simulink model "FreeFloatingNull"  (R2019a)
settings: Solver=VariableStepAuto  StartTime=0.0  StopTime=30  RelTol=1e-3
values from neighbouring files (symbols this model uses):
  deltaQdotGainArm = 1    [main.m]
  eePositionGain = 3    [main.m]
  eeVelocityGain = 1    [main.m]
  qJoints_init = [0; -0.5236; 0; -1.0472; 0; -1.0472; 0]    [main.m]
undefined symbols (not defined in the file or in its folder): sigbuilder_block, X, Y, Z
libraries: sm_lib x99, nesl_utility x51, robotcorelib x4, simulink_extras x1
(part 1 of 3)
settings Model: Creator=tori  LastModifiedBy=tori

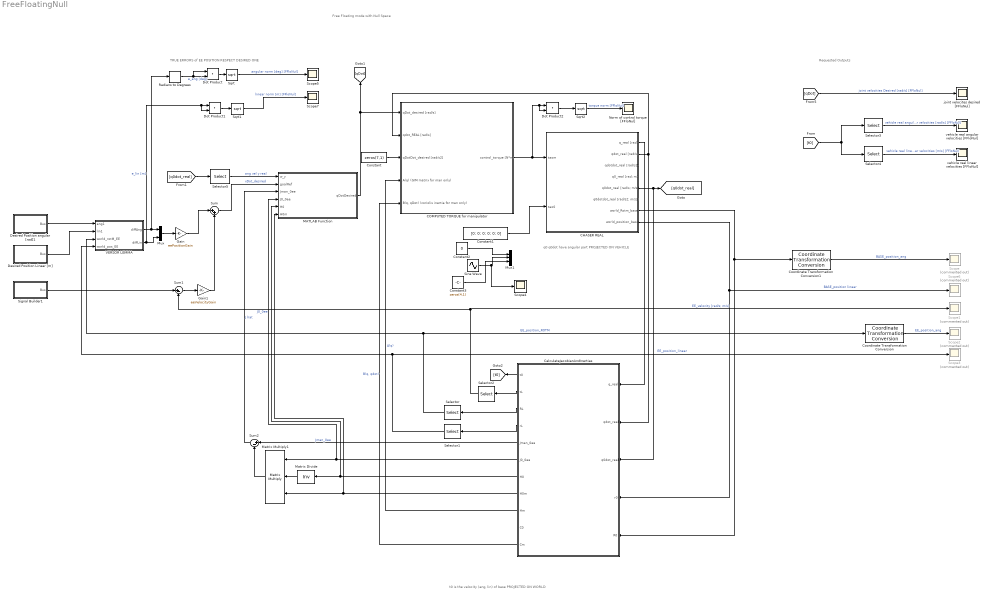
== system FreeFloatingNull ==
  note: q0 q0dot have angular part PROJECTED ON VEHICLE
  note: t0 is the velocity (ang, lin) of base PROJECTED ON WORLD
  note: TRUE ERRORS of EE POSITION RESPECT DESIRED ONE
  note: Free Floating mode with Null Space
  note: Requested Outputs
  "CHASER REAL " : Subsystem
  COMPUTED TORQUE for manipulator : Subsystem  mask{deltaQdotGainArm_int=deltaQdotGainArm}
      mask prompts: deltaQdotGainArm_int "Gain for deltaQdot"
  CalculateJacobianAndInertias : MATLAB Function  TreatAsAtomicUnit=on
  Constant : Constant  Value=zeros(7,1)
  Constant1 : Constant  Value=[0; 0; 0; 0; 0; 0]
  Constant2 : Constant  Value=0
  Constant3 : Constant  Value=zeros(4,1)
  Coordinate Transformation Conversion : robotcorelib/Coordinate Transformation Conversion  InputRepresentation=Rotation Matrix  InputEulerSequence=ZYX  ShowTrVecInputPort=on  OutputRepresentation=Euler Angles  OutputEulerSequence=ZYX  ShowTrVecOutputPort=on  SimulateUsing=Interpreted execution
      settings: SourceProductBaseCode=RO
  Coordinate Transformation Conversion1 : robotcorelib/Coordinate Transformation Conversion  InputRepresentation=Rotation Matrix  InputEulerSequence=ZYX  ShowTrVecInputPort=on  OutputRepresentation=Euler Angles  OutputEulerSequence=ZYX  ShowTrVecOutputPort=on  SimulateUsing=Interpreted execution
      settings: SourceProductBaseCode=RO
  "Desired Position Linear [m] " : Subsystem  Tag=STV Subsys  LoadFcn=sigbuilder_block('load');  StartFcn=sigbuilder_block('start');  StopFcn=sigbuilder_block('stop');  ClipboardFcn=sigbuilder_block('clipboard');  mask(Sigbuilder block){tuvar=[0:10]}
      mask help: Simulink:masks:SigbuilderBlock_MD
      mask init:
      | if ~strcmp(get_param(bdroot(gcbh),'SimulationStatus'),'stopped') tuvar = sigbuilder_block('maskInit'); end
      settings: CopyFcn=sigbuilder_block('copy');  DeleteFcn=sigbuilder_block('delete');  ModelCloseFcn=sigbuilder_block('modelClose');  PreSaveFcn=sigbuilder_block('preSave');  PauseFcn=sigbuilder_block('pause');  ContinueFcn=sigbuilder_block('continue');  NameChangeFcn=sigbuilder_block('namechange');  OpenFcn=sigbuilder_block('open',[4.5 0 1432.5 645.75 ]);  CloseFcn=sigbuilder_block('close');
      mask Display: plot(0, 0, 100, 100,[2, 2, 32, 32, 2], [68, 8, 8, 68, 68],[32, 2], [38, 38], [32, 19, 2],[53, 60, 44], [32, 17, 17, 2],[16, 16, 31, 31]);txt = getActiveGroup(gcbh);text(2, 100, txt,'verticalAlignment', 'top');
  Desired Position angular [rad]1 : Subsystem  Tag=STV Subsys  LoadFcn=sigbuilder_block('load');  StartFcn=sigbuilder_block('start');  StopFcn=sigbuilder_block('stop');  ClipboardFcn=sigbuilder_block('clipboard');  mask(Sigbuilder block){tuvar=[0:10]}
      mask help: Simulink:masks:SigbuilderBlock_MD
      mask init:
      | if ~strcmp(get_param(bdroot(gcbh),'SimulationStatus'),'stopped') tuvar = sigbuilder_block('maskInit'); end
      settings: CopyFcn=sigbuilder_block('copy');  DeleteFcn=sigbuilder_block('delete');  ModelCloseFcn=sigbuilder_block('modelClose');  PreSaveFcn=sigbuilder_block('preSave');  PauseFcn=sigbuilder_block('pause');  ContinueFcn=sigbuilder_block('continue');  NameChangeFcn=sigbuilder_block('namechange');  OpenFcn=sigbuilder_block('open',[0 0 1440 589.5 ]);  CloseFcn=sigbuilder_block('close');
      mask Display: plot(0, 0, 100, 100,[2, 2, 32, 32, 2], [68, 8, 8, 68, 68],[32, 2], [38, 38], [32, 19, 2],[53, 60, 44], [32, 17, 17, 2],[16, 16, 31, 31]);txt = getActiveGroup(gcbh);text(2, 100, txt,'verticalAlignment', 'top');
  Dot Product : DotProduct  InputSameDT=on  OutDataTypeStr=Inherit: Inherit via internal rule
  Dot Product1 : DotProduct  InputSameDT=on  OutDataTypeStr=Inherit: Inherit via internal rule
  Dot Product2 : DotProduct  InputSameDT=on  OutDataTypeStr=Inherit: Inherit via internal rule
  Gain : Gain  Gain=eePositionGain
  Gain1 : Gain  Gain=eeVelocityGain
  MATLAB Function : MATLAB Function  TreatAsAtomicUnit=on
  Matrix Divide : Product  Inputs=/  Multiplication=Matrix(*)
  Matrix Multiply1 : Product  Inputs=3  Multiplication=Matrix(*)
  Mux : Mux  Inputs=2
  Mux1 : Mux  Inputs=3
  Norm of control torque [FFloNul] : Scope
  Radians to Degrees : simulink_extras/Transformations/Radians to Degrees
  Scope{,1..3,6} (5 alike) : Scope  Commented=on
  Scope4 : Scope
  Scope5 : Scope
  Scope7 : Scope
  Selector : Selector  NumberOfDimensions=3  InputPortWidth=3  IndexOptions=Select all,Select all,Starting index (dialog)  Indices=[1 3],1,8  OutputSizes=1,1,1
  Selector1 : Selector  NumberOfDimensions=2  InputPortWidth=3  IndexOptions=Select all,Starting index (dialog)  Indices=[1 3],8  OutputSizes=1,1
  Selector2 : Selector  NumberOfDimensions=2  InputPortWidth=3  IndexOptions=Select all,Starting index (dialog)  Indices=[1 3],8  OutputSizes=1,1
  Selector3 : Selector  InputPortWidth=6  IndexOptions=Index vector (dialog)  Indices=[1 2 3]  OutputSizes=1
  Selector4 : Selector  InputPortWidth=6  IndexOptions=Index vector (dialog)  Indices=[4 5 6]  OutputSizes=1
  Selector5 : Selector  InputPortWidth=6  IndexOptions=Index vector (dialog)  Indices=[2]  OutputSizes=1
  Signal Builder1 : Subsystem  Tag=STV Subsys  LoadFcn=sigbuilder_block('load');  StartFcn=sigbuilder_block('start');  StopFcn=sigbuilder_block('stop');  ClipboardFcn=sigbuilder_block('clipboard');  mask(Sigbuilder block){tuvar=[0:10]}
      mask help: Simulink:masks:SigbuilderBlock_MD
      mask init:
      | if ~strcmp(get_param(bdroot(gcbh),'SimulationStatus'),'stopped') tuvar = sigbuilder_block('maskInit'); end
      settings: CopyFcn=sigbuilder_block('copy');  DeleteFcn=sigbuilder_block('delete');  ModelCloseFcn=sigbuilder_block('modelClose');  PreSaveFcn=sigbuilder_block('preSave');  PauseFcn=sigbuilder_block('pause');  ContinueFcn=sigbuilder_block('continue');  NameChangeFcn=sigbuilder_block('namechange');  OpenFcn=sigbuilder_block('open',[8.25 0 720 724.5 ]);  CloseFcn=sigbuilder_block('close');
      mask Display: plot(0, 0, 100, 100,[2, 2, 32, 32, 2], [68, 8, 8, 68, 68],[32, 2], [38, 38], [32, 19, 2],[53, 60, 44], [32, 17, 17, 2],[16, 16, 31, 31]);txt = getActiveGroup(gcbh);text(2, 100, txt,'verticalAlignment', 'top');
  Sine Wave : Sin  Amplitude=10  SampleTime=0
  Sqrt : Sqrt  SaturateOnIntegerOverflow=on
  Sqrt1 : Sqrt  SaturateOnIntegerOverflow=on
  Sqrt2 : Sqrt  SaturateOnIntegerOverflow=on
  Sum : Sum  Inputs=|++
  Sum1 : Sum  Inputs=|+-
  Sum2 : Sum  Inputs=|+-
  VERSOR LEMMA : MATLAB Function  TreatAsAtomicUnit=on
  "joint velocites desired [FFloNul] " : Scope
  vehicle real angular velocities [FFloNul] : Scope
  vehicle real linear velocities [FFloNul] : Scope
  wires:
  CalculateJacobianAndInertias/4(rL) -> Selector1/1
  Selector/1 -> Coordinate Transformation Conversion/1, VERSOR LEMMA/3(world_rotM_EE)  "EE_position_ROTM"
  CalculateJacobianAndInertias/9(Hm) -> COMPUTED TORQUE for manipulator/4(A(q) (GIM matrix for man only))  "A(q)"
  VERSOR LEMMA/2(diffLin) -> Dot Product1/2, Dot Product1/1, Mux/2  "e_lin [m]"
  CalculateJacobianAndInertias/11(Cm) -> COMPUTED TORQUE for manipulator/5("B(q, qDot) (coriolis inertia for man only)")  "B(q, qdot)"
  "Desired Position Linear [m] "/1(Bus) -> VERSOR LEMMA/2(lin1)
  Sum1/1 -> Gain1/1
  "CHASER REAL "/1(q_real [rad]) -> CalculateJacobianAndInertias/1(q_real)
  CalculateJacobianAndInertias/2(tL) -> Selector2/1
  Selector4/1 -> vehicle real linear velocities [FFloNul]/1  "vehicle real linear velocities [m/s] [FFloNul]"
  Sum/1 -> MATLAB Function/2(goalRef)  "xDot_desired"
  Selector3/1 -> vehicle real angular velocities [FFloNul]/1  "vehicle real angular velocities [rad/s] [FFloNul]"
  "CHASER REAL "/7("world_Rotm_base ") -> CalculateJacobianAndInertias/5(R0), Coordinate Transformation Conversion1/1
  VERSOR LEMMA/1(diffAng) -> Radians to Degrees/1, Mux/1
  Coordinate Transformation Conversion/1 -> Scope2/1  "EE_position_ang"
  Gain1/1 -> Sum/2
  Selector2/1 -> Sum1/2, Scope1/1  "EE_velocity [rad/s; m/s]"
  "CHASER REAL "/8(world_position_base) -> CalculateJacobianAndInertias/4(r0), Scope6/1  "BASE_position linear"
  [qDot] -> "joint velocites desired [FFloNul] "/1  "joint velocities Desired [rad/s] [FFloNul]"
  Signal Builder1/1(Bus) -> Sum1/1
  Mux/1 -> Gain/1
  Desired Position angular [rad]1/1(Bus) -> VERSOR LEMMA/1(ang1)
  Radians to Degrees/1 -> Dot Product/2, Dot Product/1  "e_ang [deg]"
  Constant/1 -> COMPUTED TORQUE for manipulator/3(qDotDot_desired [rad/s2])
  Selector1/1 -> Scope3/1, VERSOR LEMMA/4(world_pos_EE)  "EE_position_linear"
  Coordinate Transformation Conversion1/1 -> Scope/1  "BASE_position_ang"
  [t0] -> Selector4/1, Selector3/1
  Gain/1 -> Sum/1
  "CHASER REAL "/5(q0dot_real [rad/s; m/s]) -> [q0dot_real], CalculateJacobianAndInertias/3(q0dot_real)
  "CHASER REAL "/2(qdot_real [rad/s]) -> COMPUTED TORQUE for manipulator/2(qdot_REAL [rad/s]), CalculateJacobianAndInertias/2(qdot_real)
  CalculateJacobianAndInertias/3(RL) -> Selector/1
  Selector5/1 -> MATLAB Function/1(w_y)  "ang vel y real"
  Sqrt/1 -> Scope5/1  "angular norm [deg] [FFloNul]"
  Dot Product/1 -> Sqrt/1
  Dot Product1/1 -> Sqrt1/1
  Sqrt1/1 -> Scope7/1  "linear norm [m] [FFloNul]"
  Sqrt2/1 -> Norm of control torque [FFloNul]/1  "torque norm [FFloNul]"
  COMPUTED TORQUE for manipulator/1(control_torque [N*m]) -> Dot Product2/2, Dot Product2/1, "CHASER REAL "/1("taom ")
  Dot Product2/1 -> Sqrt2/1
  Sine Wave/1 -> Scope4/1, Mux1/2
  Constant2/1 -> Mux1/1
  Constant3/1 -> Mux1/3
  Sum2/1 -> MATLAB Function/3(Jman_0ee)  "J hat"
  CalculateJacobianAndInertias/5(Jman_0ee) -> Sum2/1  "Jman_0ee"
  CalculateJacobianAndInertias/7(H0) -> MATLAB Function/5(H0), Matrix Divide/1
  Matrix Divide/1 -> Matrix Multiply1/2
  CalculateJacobianAndInertias/8(H0m) -> MATLAB Function/6(H0m), Matrix Multiply1/3
  Matrix Multiply1/1 -> Sum2/2
  MATLAB Function/1(qDotDesired) -> COMPUTED TORQUE for manipulator/1(qDot_desired [rad/s]), [qDot]
  CalculateJacobianAndInertias/1(t0) -> [t0]
  CalculateJacobianAndInertias/6(J0_0ee) -> MATLAB Function/4(J0_0ee), Matrix Multiply1/1  "J0_0ee"
  [q0dot_real] -> Selector5/1
  Constant1/1 -> "CHASER REAL "/2(tao0)

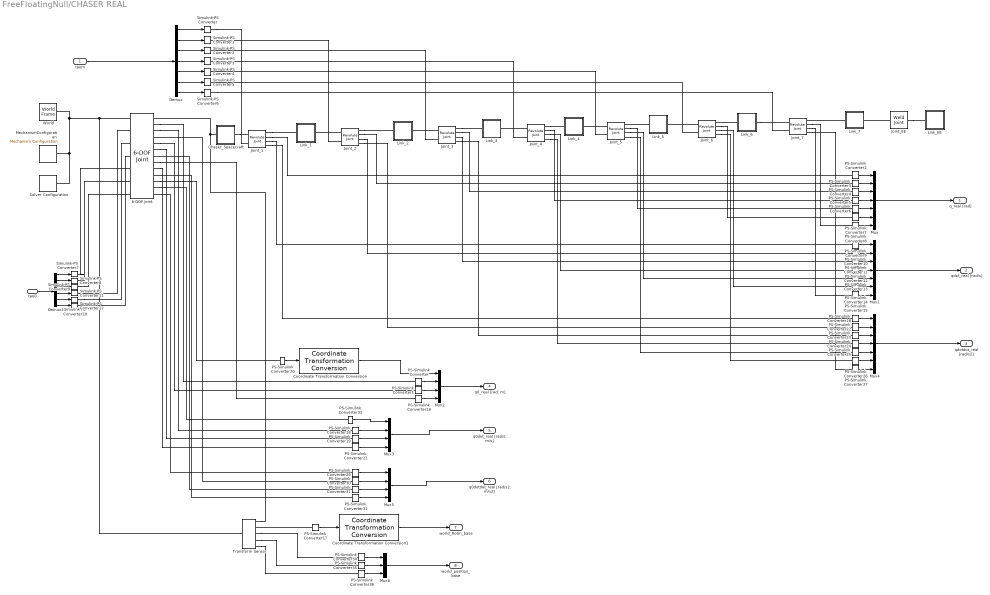
== system FreeFloatingNull/CHASER REAL  ==
  "taom " : Inport
  tao0 : Inport  Port=2
  6-DOF Joint : sm_lib/Joints/6-DOF Joint  SenseConstraintForce=off  SenseConstraintForceX=off  SenseConstraintForceY=off  SenseConstraintForceZ=off  SenseConstraintTorque=off  SenseConstraintTorqueX=off  SenseConstraintTorqueY=off  SenseConstraintTorqueZ=off  SenseTotalForce=off  SenseTotalForceX=off  SenseTotalForceY=off  SenseTotalForceZ=off  SenseTotalTorque=off  SenseTotalTorqueX=off  SenseTotalTorqueY=off  SenseTotalTorqueZ=off  CompositeWrenchDir=FollowerOnBase  CompositeWrenchFrame=BaseFrame  PxEquilibriumPosition=0  PxEquilibriumPositionUnits=m  PxSpringStiffness=0  PxSpringStiffnessUnits=N/m  PxDampingCoefficient=0  PxDampingCoefficientUnits=N/(m/s)  PxTorqueActuationMode=InputTorque  PxMotionActuationMode=ComputedMotion  PxSensePosition=on  PxSenseVelocity=on  PxSenseAcceleration=on  PxSenseTorqueForce=off  PxSenseLowerLimitTorqueForce=off  PxSenseUpperLimitTorqueForce=off  PxLowerLimitSpecify=off  PxLowerLimitBound=-1  PxLowerLimitBoundUnits=m  PxLowerLimitStiffness=1e6  PxLowerLimitStiffnessUnits=N/m  PxLowerLimitDamping=1e3  PxLowerLimitDampingUnits=N/(m/s)  PxLowerLimitTransitionRegionWidth=1e-4  PxLowerLimitTransitionRegionWidthUnits=m  PxUpperLimitSpecify=off  PxUpperLimitBound=1  PxUpperLimitBoundUnits=m  PxUpperLimitStiffness=1e6  PxUpperLimitStiffnessUnits=N/m  PxUpperLimitDamping=1e3  PxUpperLimitDampingUnits=N/(m/s)  PxUpperLimitTransitionRegionWidth=1e-4  PxUpperLimitTransitionRegionWidthUnits=m  PxPositionTargetSpecify=off  PxPositionTargetPriority=High  PxPositionTargetValue=0  PxPositionTargetValueUnits=m  PxVelocityTargetSpecify=off  PxVelocityTargetPriority=High  PxVelocityTargetValue=0  PxVelocityTargetValueUnits=m/s  PyEquilibriumPosition=0  PyEquilibriumPositionUnits=m  PySpringStiffness=0  PySpringStiffnessUnits=N/m  PyDampingCoefficient=0  PyDampingCoefficientUnits=N/(m/s)  PyTorqueActuationMode=InputTorque  PyMotionActuationMode=ComputedMotion  PySensePosition=on  PySenseVelocity=on  PySenseAcceleration=on  PySenseTorqueForce=off  PySenseLowerLimitTorqueForce=off  PySenseUpperLimitTorqueForce=off  PyLowerLimitSpecify=off  PyLowerLimitBound=-1  PyLowerLimitBoundUnits=m  PyLowerLimitStiffness=1e6  PyLowerLimitStiffnessUnits=N/m  PyLowerLimitDamping=1e3  PyLowerLimitDampingUnits=N/(m/s)  PyLowerLimitTransitionRegionWidth=1e-4  PyLowerLimitTransitionRegionWidthUnits=m  PyUpperLimitSpecify=off  PyUpperLimitBound=1  PyUpperLimitBoundUnits=m  PyUpperLimitStiffness=1e6  PyUpperLimitStiffnessUnits=N/m  PyUpperLimitDamping=1e3  PyUpperLimitDampingUnits=N/(m/s)  PyUpperLimitTransitionRegionWidth=1e-4  PyUpperLimitTransitionRegionWidthUnits=m  PyPositionTargetSpecify=off  PyPositionTargetPriority=High  PyPositionTargetValue=0  PyPositionTargetValueUnits=m  PyVelocityTargetSpecify=off  PyVelocityTargetPriority=High  PyVelocityTargetValue=0  PyVelocityTargetValueUnits=m/s  PzEquilibriumPosition=0  PzEquilibriumPositionUnits=m  PzSpringStiffness=0  PzSpringStiffnessUnits=N/m  PzDampingCoefficient=0  PzDampingCoefficientUnits=N/(m/s)  PzTorqueActuationMode=InputTorque  PzMotionActuationMode=ComputedMotion  PzSensePosition=on  PzSenseVelocity=on  PzSenseAcceleration=on  PzSenseTorqueForce=off  PzSenseLowerLimitTorqueForce=off  PzSenseUpperLimitTorqueForce=off  PzLowerLimitSpecify=off  PzLowerLimitBound=-1  PzLowerLimitBoundUnits=m  PzLowerLimitStiffness=1e6  PzLowerLimitStiffnessUnits=N/m  PzLowerLimitDamping=1e3  PzLowerLimitDampingUnits=N/(m/s)  PzLowerLimitTransitionRegionWidth=1e-4  PzLowerLimitTransitionRegionWidthUnits=m  PzUpperLimitSpecify=off  PzUpperLimitBound=1  PzUpperLimitBoundUnits=m  PzUpperLimitStiffness=1e6  PzUpperLimitStiffnessUnits=N/m  PzUpperLimitDamping=1e3  PzUpperLimitDampingUnits=N/(m/s)  PzUpperLimitTransitionRegionWidth=1e-4  PzUpperLimitTransitionRegionWidthUnits=m  PzPositionTargetSpecify=off  PzPositionTargetPriority=High  PzPositionTargetValue=0  PzPositionTargetValueUnits=m  PzVelocityTargetSpecify=off  PzVelocityTargetPriority=High  PzVelocityTargetValue=0  PzVelocityTargetValueUnits=m/s  SphDefPosRotationMethod=None  SphDefPosRotationAngleUnits=deg  SphDefPosRotationStandardAxis=+Z  SphDefPosRotationAngle=0.0  SphDefPosRotationArbitraryAxis=[0 0 1]  SphDefPosFollAlignAxisA=+X  SphDefPosBaseAlignAxisA=+Y  SphDefPosFollAlignAxisB=+Y  SphDefPosBaseAlignAxisB=+Z  SphDefPosRotationSequenceAxes=FollowerAxes  SphDefPosRotationSequence=XYX  SphDefPosRotationSequenceAngles=[0 0 0]  SphDefPosRotationSequenceAnglesUnits=deg  SphDefPosRotationMatrix=[1 0 0; 0 1 0; 0 0 1]  SphEqPosRotationMethod=None  SphEqPosRotationAngleUnits=deg  SphEqPosRotationStandardAxis=+Z  SphEqPosRotationAngle=0.0  SphEqPosRotationArbitraryAxis=[0 0 1]  SphEqPosFollAlignAxisA=+X  SphEqPosBaseAlignAxisA=+Y  SphEqPosFollAlignAxisB=+Y  SphEqPosBaseAlignAxisB=+Z  SphEqPosRotationSequenceAxes=FollowerAxes  SphEqPosRotationSequence=XYX  SphEqPosRotationSequenceAngles=[0 0 0]  SphEqPosRotationSequenceAnglesUnits=deg  SphEqPosRotationMatrix=[1 0 0; 0 1 0; 0 0 1]  SphSpringStiffness=0  SphSpringStiffnessUnits=N*m/deg  SphDampingCoefficient=0  SphDampingCoefficientUnits=N*m/(deg/s)  SphActuateTorqueX=on  SphActuateTorqueY=on  SphActuateTorqueZ=on  SphActuateTorque=off  SphTorqueActuationMode=InputTorque  SphMotionActuationMode=ComputedMotion  SphActuationFrame=FollowerFrame  SphSensePosition=on  SphSenseVelocityX=off  SphSenseVelocityY=off  SphSenseVelocityZ=off  SphSenseVelocity=on  SphSenseAccelerationX=off  SphSenseAccelerationY=off  SphSenseAccelerationZ=off  SphSenseAcceleration=on  SphSenseTorqueX=off  SphSenseTorqueY=off  SphSenseTorqueZ=off  SphSenseTorqueForce=off  SphSenseLowerLimitTorqueMag=off  SphSenseUpperLimitTorqueMag=off  SphSensingFrame=FollowerFrame  SphLowerLimitSpecify=off  SphLowerLimitBound=15  SphLowerLimitBoundUnits=deg  SphLowerLimitStiffness=1e4  SphLowerLimitStiffnessUnits=N*m/deg  SphLowerLimitDamping=10  SphLowerLimitDampingUnits=N*m/(deg/s)  SphLowerLimitTransitionRegionWidth=0.1  SphLowerLimitTransitionRegionWidthUnits=deg  SphUpperLimitSpecify=off  SphUpperLimitBound=45  SphUpperLimitBoundUnits=deg  SphUpperLimitStiffness=1e4  SphUpperLimitStiffnessUnits=N*m/deg  SphUpperLimitDamping=10  SphUpperLimitDampingUnits=N*m/(deg/s)  SphUpperLimitTransitionRegionWidth=0.1  SphUpperLimitTransitionRegionWidthUnits=deg  SphPositionTargetRotationMethod=None  SphPositionTargetRotationAngleUnits=deg  SphPositionTargetRotationStandardAxis=+Z  SphPositionTargetRotationAngle=0.0  SphPositionTargetRotationArbitraryAxis=[0 0 1]  SphPositionTargetFollAlignAxisA=+X  SphPositionTargetBaseAlignAxisA=+Y  SphPositionTargetFollAlignAxisB=+Y  SphPositionTargetBaseAlignAxisB=+Z  SphPositionTargetRotationSequenceAxes=FollowerAxes  SphPositionTargetRotationSequence=XYX  SphPositionTargetRotationSequenceAngles=[0 0 0]  SphPositionTargetRotationSequenceAnglesUnits=deg  SphPositionTargetRotationMatrix=[1 0 0; 0 1 0; 0 0 1]  SphPositionTargetSpecify=off  SphPositionTargetPriority=High  SphVelocityTargetValue=[0 0 0]  SphVelocityTargetValueUnits=deg/s  SphVelocityTargetSpecify=off  SphVelocityTargetPriority=High  SphVelocityTargetInFollowerFrame=on
  Chaser_Spacecraft : Subsystem
  Coordinate Transformation Conversion : robotcorelib/Coordinate Transformation Conversion  InputRepresentation=Quaternion  InputEulerSequence=ZYX  ShowTrVecInputPort=on  OutputRepresentation=Euler Angles  OutputEulerSequence=ZYX  ShowTrVecOutputPort=on  SimulateUsing=Interpreted execution
      settings: SourceProductBaseCode=RO
  Coordinate Transformation Conversion1 : robotcorelib/Coordinate Transformation Conversion  InputRepresentation=Quaternion  InputEulerSequence=ZYX  ShowTrVecInputPort=on  OutputRepresentation=Rotation Matrix  OutputEulerSequence=ZYX  ShowTrVecOutputPort=on  SimulateUsing=Interpreted execution
      settings: SourceProductBaseCode=RO
  Demux : Demux  Outputs=7
  Demux1 : Demux  Outputs=6
  Joint_1 : sm_lib/Joints/Revolute Joint  SenseConstraintForce=off  SenseConstraintForceX=off  SenseConstraintForceY=off  SenseConstraintForceZ=off  SenseConstraintTorque=off  SenseConstraintTorqueX=off  SenseConstraintTorqueY=off  SenseConstraintTorqueZ=off  SenseTotalForce=off  SenseTotalForceX=off  SenseTotalForceY=off  SenseTotalForceZ=off  SenseTotalTorque=off  SenseTotalTorqueX=off  SenseTotalTorqueY=off  SenseTotalTorqueZ=off  CompositeWrenchDir=FollowerOnBase  CompositeWrenchFrame=BaseFrame  EquilibriumPosition=0  EquilibriumPositionUnits=deg  SpringStiffness=0  SpringStiffnessUnits=N*m/deg  DampingCoefficient=0  DampingCoefficientUnits=m^2*kg/s/rad  TorqueActuationMode=InputTorque  MotionActuationMode=ComputedMotion  SensePosition=on  SenseVelocity=on  SenseAcceleration=on  SenseTorqueForce=off  SenseLowerLimitTorqueForce=off  SenseUpperLimitTorqueForce=off  LowerLimitSpecify=off  LowerLimitBound=-90  LowerLimitBoundUnits=deg  LowerLimitStiffness=1e4  LowerLimitStiffnessUnits=N*m/deg  LowerLimitDamping=10  LowerLimitDampingUnits=N*m/(deg/s)  LowerLimitTransitionRegionWidth=0.1  LowerLimitTransitionRegionWidthUnits=deg  UpperLimitSpecify=off  UpperLimitBound=90  UpperLimitBoundUnits=deg  UpperLimitStiffness=1e4  UpperLimitStiffnessUnits=N*m/deg  UpperLimitDamping=10  UpperLimitDampingUnits=N*m/(deg/s)  UpperLimitTransitionRegionWidth=0.1  UpperLimitTransitionRegionWidthUnits=deg  PositionTargetSpecify=on  PositionTargetPriority=High  PositionTargetValue=qJoints_init(1)  PositionTargetValueUnits=rad  VelocityTargetSpecify=off  VelocityTargetPriority=High  VelocityTargetValue=0  VelocityTargetValueUnits=deg/s
  Joint_2 : sm_lib/Joints/Revolute Joint  SenseConstraintForce=off  SenseConstraintForceX=off  SenseConstraintForceY=off  SenseConstraintForceZ=off  SenseConstraintTorque=off  SenseConstraintTorqueX=off  SenseConstraintTorqueY=off  SenseConstraintTorqueZ=off  SenseTotalForce=off  SenseTotalForceX=off  SenseTotalForceY=off  SenseTotalForceZ=off  SenseTotalTorque=off  SenseTotalTorqueX=off  SenseTotalTorqueY=off  SenseTotalTorqueZ=off  CompositeWrenchDir=FollowerOnBase  CompositeWrenchFrame=BaseFrame  EquilibriumPosition=0  EquilibriumPositionUnits=deg  SpringStiffness=0  SpringStiffnessUnits=N*m/deg  DampingCoefficient=0  DampingCoefficientUnits=m^2*kg/s/rad  TorqueActuationMode=InputTorque  MotionActuationMode=ComputedMotion  SensePosition=on  SenseVelocity=on  SenseAcceleration=on  SenseTorqueForce=off  SenseLowerLimitTorqueForce=off  SenseUpperLimitTorqueForce=off  LowerLimitSpecify=off  LowerLimitBound=-90  LowerLimitBoundUnits=deg  LowerLimitStiffness=1e4  LowerLimitStiffnessUnits=N*m/deg  LowerLimitDamping=10  LowerLimitDampingUnits=N*m/(deg/s)  LowerLimitTransitionRegionWidth=0.1  LowerLimitTransitionRegionWidthUnits=deg  UpperLimitSpecify=off  UpperLimitBound=90  UpperLimitBoundUnits=deg  UpperLimitStiffness=1e4  UpperLimitStiffnessUnits=N*m/deg  UpperLimitDamping=10  UpperLimitDampingUnits=N*m/(deg/s)  UpperLimitTransitionRegionWidth=0.1  UpperLimitTransitionRegionWidthUnits=deg  PositionTargetSpecify=on  PositionTargetPriority=High  PositionTargetValue=qJoints_init(2)  PositionTargetValueUnits=rad  VelocityTargetSpecify=off  VelocityTargetPriority=High  VelocityTargetValue=0  VelocityTargetValueUnits=deg/s
  Joint_3 : sm_lib/Joints/Revolute Joint  SenseConstraintForce=off  SenseConstraintForceX=off  SenseConstraintForceY=off  SenseConstraintForceZ=off  SenseConstraintTorque=off  SenseConstraintTorqueX=off  SenseConstraintTorqueY=off  SenseConstraintTorqueZ=off  SenseTotalForce=off  SenseTotalForceX=off  SenseTotalForceY=off  SenseTotalForceZ=off  SenseTotalTorque=off  SenseTotalTorqueX=off  SenseTotalTorqueY=off  SenseTotalTorqueZ=off  CompositeWrenchDir=FollowerOnBase  CompositeWrenchFrame=BaseFrame  EquilibriumPosition=0  EquilibriumPositionUnits=deg  SpringStiffness=0  SpringStiffnessUnits=N*m/deg  DampingCoefficient=0  DampingCoefficientUnits=m^2*kg/s/rad  TorqueActuationMode=InputTorque  MotionActuationMode=ComputedMotion  SensePosition=on  SenseVelocity=on  SenseAcceleration=on  SenseTorqueForce=off  SenseLowerLimitTorqueForce=off  SenseUpperLimitTorqueForce=off  LowerLimitSpecify=off  LowerLimitBound=-90  LowerLimitBoundUnits=deg  LowerLimitStiffness=1e4  LowerLimitStiffnessUnits=N*m/deg  LowerLimitDamping=10  LowerLimitDampingUnits=N*m/(deg/s)  LowerLimitTransitionRegionWidth=0.1  LowerLimitTransitionRegionWidthUnits=deg  UpperLimitSpecify=off  UpperLimitBound=90  UpperLimitBoundUnits=deg  UpperLimitStiffness=1e4  UpperLimitStiffnessUnits=N*m/deg  UpperLimitDamping=10  UpperLimitDampingUnits=N*m/(deg/s)  UpperLimitTransitionRegionWidth=0.1  UpperLimitTransitionRegionWidthUnits=deg  PositionTargetSpecify=on  PositionTargetPriority=High  PositionTargetValue=qJoints_init(3)  PositionTargetValueUnits=rad  VelocityTargetSpecify=off  VelocityTargetPriority=High  VelocityTargetValue=0  VelocityTargetValueUnits=deg/s
  Joint_4 : sm_lib/Joints/Revolute Joint  SenseConstraintForce=off  SenseConstraintForceX=off  SenseConstraintForceY=off  SenseConstraintForceZ=off  SenseConstraintTorque=off  SenseConstraintTorqueX=off  SenseConstraintTorqueY=off  SenseConstraintTorqueZ=off  SenseTotalForce=off  SenseTotalForceX=off  SenseTotalForceY=off  SenseTotalForceZ=off  SenseTotalTorque=off  SenseTotalTorqueX=off  SenseTotalTorqueY=off  SenseTotalTorqueZ=off  CompositeWrenchDir=FollowerOnBase  CompositeWrenchFrame=BaseFrame  EquilibriumPosition=0  EquilibriumPositionUnits=deg  SpringStiffness=0  SpringStiffnessUnits=N*m/deg  DampingCoefficient=0  DampingCoefficientUnits=m^2*kg/s/rad  TorqueActuationMode=InputTorque  MotionActuationMode=ComputedMotion  SensePosition=on  SenseVelocity=on  SenseAcceleration=on  SenseTorqueForce=off  SenseLowerLimitTorqueForce=off  SenseUpperLimitTorqueForce=off  LowerLimitSpecify=off  LowerLimitBound=-90  LowerLimitBoundUnits=deg  LowerLimitStiffness=1e4  LowerLimitStiffnessUnits=N*m/deg  LowerLimitDamping=10  LowerLimitDampingUnits=N*m/(deg/s)  LowerLimitTransitionRegionWidth=0.1  LowerLimitTransitionRegionWidthUnits=deg  UpperLimitSpecify=off  UpperLimitBound=90  UpperLimitBoundUnits=deg  UpperLimitStiffness=1e4  UpperLimitStiffnessUnits=N*m/deg  UpperLimitDamping=10  UpperLimitDampingUnits=N*m/(deg/s)  UpperLimitTransitionRegionWidth=0.1  UpperLimitTransitionRegionWidthUnits=deg  PositionTargetSpecify=on  PositionTargetPriority=High  PositionTargetValue=qJoints_init(4)  PositionTargetValueUnits=rad  VelocityTargetSpecify=off  VelocityTargetPriority=High  VelocityTargetValue=0  VelocityTargetValueUnits=deg/s
  Joint_5 : sm_lib/Joints/Revolute Joint  SenseConstraintForce=off  SenseConstraintForceX=off  SenseConstraintForceY=off  SenseConstraintForceZ=off  SenseConstraintTorque=off  SenseConstraintTorqueX=off  SenseConstraintTorqueY=off  SenseConstraintTorqueZ=off  SenseTotalForce=off  SenseTotalForceX=off  SenseTotalForceY=off  SenseTotalForceZ=off  SenseTotalTorque=off  SenseTotalTorqueX=off  SenseTotalTorqueY=off  SenseTotalTorqueZ=off  CompositeWrenchDir=FollowerOnBase  CompositeWrenchFrame=BaseFrame  EquilibriumPosition=0  EquilibriumPositionUnits=deg  SpringStiffness=0  SpringStiffnessUnits=N*m/deg  DampingCoefficient=0  DampingCoefficientUnits=m^2*kg/s/rad  TorqueActuationMode=InputTorque  MotionActuationMode=ComputedMotion  SensePosition=on  SenseVelocity=on  SenseAcceleration=on  SenseTorqueForce=off  SenseLowerLimitTorqueForce=off  SenseUpperLimitTorqueForce=off  LowerLimitSpecify=off  LowerLimitBound=-90  LowerLimitBoundUnits=deg  LowerLimitStiffness=1e4  LowerLimitStiffnessUnits=N*m/deg  LowerLimitDamping=10  LowerLimitDampingUnits=N*m/(deg/s)  LowerLimitTransitionRegionWidth=0.1  LowerLimitTransitionRegionWidthUnits=deg  UpperLimitSpecify=off  UpperLimitBound=90  UpperLimitBoundUnits=deg  UpperLimitStiffness=1e4  UpperLimitStiffnessUnits=N*m/deg  UpperLimitDamping=10  UpperLimitDampingUnits=N*m/(deg/s)  UpperLimitTransitionRegionWidth=0.1  UpperLimitTransitionRegionWidthUnits=deg  PositionTargetSpecify=on  PositionTargetPriority=High  PositionTargetValue=qJoints_init(5)  PositionTargetValueUnits=rad  VelocityTargetSpecify=off  VelocityTargetPriority=High  VelocityTargetValue=0  VelocityTargetValueUnits=deg/s
  Joint_6 : sm_lib/Joints/Revolute Joint  SenseConstraintForce=off  SenseConstraintForceX=off  SenseConstraintForceY=off  SenseConstraintForceZ=off  SenseConstraintTorque=off  SenseConstraintTorqueX=off  SenseConstraintTorqueY=off  SenseConstraintTorqueZ=off  SenseTotalForce=off  SenseTotalForceX=off  SenseTotalForceY=off  SenseTotalForceZ=off  SenseTotalTorque=off  SenseTotalTorqueX=off  SenseTotalTorqueY=off  SenseTotalTorqueZ=off  CompositeWrenchDir=FollowerOnBase  CompositeWrenchFrame=BaseFrame  EquilibriumPosition=0  EquilibriumPositionUnits=deg  SpringStiffness=0  SpringStiffnessUnits=N*m/deg  DampingCoefficient=0  DampingCoefficientUnits=m^2*kg/s/rad  TorqueActuationMode=InputTorque  MotionActuationMode=ComputedMotion  SensePosition=on  SenseVelocity=on  SenseAcceleration=on  SenseTorqueForce=off  SenseLowerLimitTorqueForce=off  SenseUpperLimitTorqueForce=off  LowerLimitSpecify=off  LowerLimitBound=-90  LowerLimitBoundUnits=deg  LowerLimitStiffness=1e4  LowerLimitStiffnessUnits=N*m/deg  LowerLimitDamping=10  LowerLimitDampingUnits=N*m/(deg/s)  LowerLimitTransitionRegionWidth=0.1  LowerLimitTransitionRegionWidthUnits=deg  UpperLimitSpecify=off  UpperLimitBound=90  UpperLimitBoundUnits=deg  UpperLimitStiffness=1e4  UpperLimitStiffnessUnits=N*m/deg  UpperLimitDamping=10  UpperLimitDampingUnits=N*m/(deg/s)  UpperLimitTransitionRegionWidth=0.1  UpperLimitTransitionRegionWidthUnits=deg  PositionTargetSpecify=on  PositionTargetPriority=High  PositionTargetValue=qJoints_init(6)  PositionTargetValueUnits=rad  VelocityTargetSpecify=off  VelocityTargetPriority=High  VelocityTargetValue=0  VelocityTargetValueUnits=deg/s
  Joint_7 : sm_lib/Joints/Revolute Joint  SenseConstraintForce=off  SenseConstraintForceX=off  SenseConstraintForceY=off  SenseConstraintForceZ=off  SenseConstraintTorque=off  SenseConstraintTorqueX=off  SenseConstraintTorqueY=off  SenseConstraintTorqueZ=off  SenseTotalForce=off  SenseTotalForceX=off  SenseTotalForceY=off  SenseTotalForceZ=off  SenseTotalTorque=off  SenseTotalTorqueX=off  SenseTotalTorqueY=off  SenseTotalTorqueZ=off  CompositeWrenchDir=FollowerOnBase  CompositeWrenchFrame=BaseFrame  EquilibriumPosition=0  EquilibriumPositionUnits=deg  SpringStiffness=0  SpringStiffnessUnits=N*m/deg  DampingCoefficient=0  DampingCoefficientUnits=m^2*kg/s/rad  TorqueActuationMode=InputTorque  MotionActuationMode=ComputedMotion  SensePosition=on  SenseVelocity=on  SenseAcceleration=on  SenseTorqueForce=off  SenseLowerLimitTorqueForce=off  SenseUpperLimitTorqueForce=off  LowerLimitSpecify=off  LowerLimitBound=-90  LowerLimitBoundUnits=deg  LowerLimitStiffness=1e4  LowerLimitStiffnessUnits=N*m/deg  LowerLimitDamping=10  LowerLimitDampingUnits=N*m/(deg/s)  LowerLimitTransitionRegionWidth=0.1  LowerLimitTransitionRegionWidthUnits=deg  UpperLimitSpecify=off  UpperLimitBound=90  UpperLimitBoundUnits=deg  UpperLimitStiffness=1e4  UpperLimitStiffnessUnits=N*m/deg  UpperLimitDamping=10  UpperLimitDampingUnits=N*m/(deg/s)  UpperLimitTransitionRegionWidth=0.1  UpperLimitTransitionRegionWidthUnits=deg  PositionTargetSpecify=on  PositionTargetPriority=High  PositionTargetValue=qJoints_init(7)  PositionTargetValueUnits=rad  VelocityTargetSpecify=off  VelocityTargetPriority=High  VelocityTargetValue=0  VelocityTargetValueUnits=deg/s
  Joint_EE : sm_lib/Joints/Weld Joint  SenseConstraintForce=off  SenseConstraintForceX=off  SenseConstraintForceY=off  SenseConstraintForceZ=off  SenseConstraintTorque=off  SenseConstraintTorqueX=off  SenseConstraintTorqueY=off  SenseConstraintTorqueZ=off  SenseTotalForce=off  SenseTotalForceX=off  SenseTotalForceY=off  SenseTotalForceZ=off  SenseTotalTorque=off  SenseTotalTorqueX=off  SenseTotalTorqueY=off  SenseTotalTorqueZ=off  CompositeWrenchDir=FollowerOnBase  CompositeWrenchFrame=BaseFrame
  Link_1 : Subsystem
  Link_2 : Subsystem
  Link_3 : Subsystem
  Link_4 : Subsystem
  Link_5 : Subsystem
  Link_6 : Subsystem
  Link_7 : Subsystem
  Link_EE : Subsystem
  MechanismConfiguration : sm_lib/Utilities/Mechanism Configuration  UniformGravity=None  GravityVector=[0 0 1]  GravityUnits=m/s^2  LinearizationDelta=0.001
  Mux : Mux  Inputs=7
  Mux1 : Mux  Inputs=7
  Mux2 : Mux
  Mux3 : Mux
  Mux4 : Mux  Inputs=7
  Mux5 : Mux
  Mux6 : Mux  Inputs=3
  PS-Simulink Converter{,1..36} (37 alike) : nesl_utility/PS-Simulink Converter  PhysicalDomain=network_engine_domain  SubClassName=ps_output  LeftPortType=input  RightPortType=output  PseudoPeriodic=off  Frequencies=[]  Unit=1  AffineConversion=off
  Simulink-PS Converter{,1..9} (10 alike) : nesl_utility/Simulink-PS Converter  PhysicalDomain=network_engine_domain  SubClassName=ps_input  LeftPortType=input  RightPortType=output  PseudoPeriodic=off  Frequencies=[]  NoiseDistribution=none  NoiseParameters=[]  Unit=N*m  AffineConversion=off  FilteringAndDerivatives=provide  SimscapeFilterOrder=1  InputFilterTimeConstant=0.001  UdotUserProvided=0
  Simulink-PS Converter10 : nesl_utility/Simulink-PS Converter  PhysicalDomain=network_engine_domain  SubClassName=ps_input  LeftPortType=input  RightPortType=output  PseudoPeriodic=off  Frequencies=[]  NoiseDistribution=none  NoiseParameters=[]  Unit=N  AffineConversion=off  FilteringAndDerivatives=provide  SimscapeFilterOrder=1  InputFilterTimeConstant=0.001  UdotUserProvided=0
  Simulink-PS Converter11 : nesl_utility/Simulink-PS Converter  PhysicalDomain=network_engine_domain  SubClassName=ps_input  LeftPortType=input  RightPortType=output  PseudoPeriodic=off  Frequencies=[]  NoiseDistribution=none  NoiseParameters=[]  Unit=N  AffineConversion=off  FilteringAndDerivatives=provide  SimscapeFilterOrder=1  InputFilterTimeConstant=0.001  UdotUserProvided=0
  Simulink-PS Converter12 : nesl_utility/Simulink-PS Converter  PhysicalDomain=network_engine_domain  SubClassName=ps_input  LeftPortType=input  RightPortType=output  PseudoPeriodic=off  Frequencies=[]  NoiseDistribution=none  NoiseParameters=[]  Unit=N  AffineConversion=off  FilteringAndDerivatives=provide  SimscapeFilterOrder=1  InputFilterTimeConstant=0.001  UdotUserProvided=0
  Solver Configuration : nesl_utility/Solver Configuration  PhysicalDomain=network_engine_domain  SubClassName=solver  LeftPortType=input  RightPortType=generic  Tones=[]  Harmonics=[]  SimulateNoise=off  Profile=off  UseLocalSampling=off  EnableSwitchedLinearOptims=on  FrequencyDomain=off  UseCCode=off  RelTol=0.001  AbsTol=1e-06  MinStep=1e-09  ToWorkspace=off  RevertToSquareIcSolve=off  NumHomotopyIterations=100  PhasorMode=off  PhasorModeNumHarmonics=1  DoDC=off  ResidualTolerance=1e-09  UseLocalSolver=off  LocalSolverChoice=NE_BACKWARD_EULER_ADVANCER  LocalSolverSampleTime=0.001  DoFixedCost=off  MaxNonlinIter=3  MaxModeIter=2  LinearAlgebra=auto  EquationFormulation=NE_TIME_EF  DelaysMemoryBudget=1024  AutomaticFiltering=on  FilteringTimeConstant=0.001  PartitionStorageMethod=AS_NEEDED  PartitionMemoryBudget=1024  PartitionMethod=ROBUST
  Transform Sensor : sm_lib/Frames and Transforms/Transform Sensor  MeasurementFrame=World  SenseAngle=off  SenseAxis=off  SenseAngle1=off  SenseAngle2=off  SenseAngle3=off  SenseQ=on  SenseR=off  SenseOmegaX=off  SenseOmegaY=off  SenseOmegaZ=off  SenseOmega1=off  SenseOmega2=off  SenseOmega3=off  SenseQDot=off  SenseRDot=off  SenseAlphaX=off  SenseAlphaY=off  SenseAlphaZ=off  SenseAlpha1=off  SenseAlpha2=off  SenseAlpha3=off  SenseQDDot=off  SenseRDDot=off  SenseX=on  SenseY=on  SenseZ=on  SenseRad=off  SenseAzim=off  SenseDist=off  SenseInc=off  SenseXDot=off  SenseYDot=off  SenseZDot=off  SenseRadDot=off  SenseAzimDot=off  SenseDistDot=off  SenseIncDot=off  SenseXDDot=off  SenseYDDot=off  SenseZDDot=off  SenseRadDDot=off  SenseAzimDDot=off  SenseDistDDot=off  SenseIncDDot=off
  World : sm_lib/Frames and Transforms/World Frame
  q_real [rad] : Outport
  qdot_real [rad/s] : Outport  Port=2
  qdotdot_real [rad/s2] : Outport  Port=3
  q0_real [rad; m] : Outport  Port=4
  q0dot_real [rad/s; m/s] : Outport  Port=5
  q0dotdot_real [rad/s2; m/s2] : Outport  Port=6
  "world_Rotm_base " : Outport  Port=7
  world_position_base : Outport  Port=8
  wires:
  PS-Simulink Converter26/1 -> Mux4/6
  PS-Simulink Converter7/1 -> Mux/6
  PS-Simulink Converter/1 -> Mux2/2
  PS-Simulink Converter12/1 -> Mux1/4
  PS-Simulink Converter8/1 -> Mux/7
  "taom "/1 -> Demux/1
  Coordinate Transformation Conversion/1 -> Mux2/1
  Mux5/1 -> q0dotdot_real [rad/s2; m/s2]/1
  PS-Simulink Converter30/1 -> Mux5/2
  PS-Simulink Converter33/1 -> Mux3/1
  PS-Simulink Converter32/1 -> Mux5/4
  Mux/1 -> q_real [rad]/1
  PS-Simulink Converter29/1 -> Mux5/1
  PS-Simulink Converter21/1 -> Mux3/4
  PS-Simulink Converter11/1 -> Mux1/3
  Demux/2 -> Simulink-PS Converter1/1
  PS-Simulink Converter20/1 -> Coordinate Transformation Conversion/1
  PS-Simulink Converter25/1 -> Mux4/5
  PS-Simulink Converter23/1 -> Mux4/3
  PS-Simulink Converter10/1 -> Mux1/2
  Mux3/1 -> q0dot_real [rad/s; m/s]/1
  PS-Simulink Converter14/1 -> Mux1/6
  PS-Simulink Converter2/1 -> Mux/1
  PS-Simulink Converter19/1 -> Mux3/3
  PS-Simulink Converter4/1 -> Mux/3
  PS-Simulink Converter3/1 -> Mux/2
  PS-Simulink Converter6/1 -> Mux/5
  Demux/1 -> Simulink-PS Converter/1
  PS-Simulink Converter5/1 -> Mux/4
  PS-Simulink Converter22/1 -> Mux4/2
  Mux2/1 -> q0_real [rad; m]/1
  PS-Simulink Converter31/1 -> Mux5/3
  PS-Simulink Converter18/1 -> Mux3/2
  Mux1/1 -> qdot_real [rad/s]/1
  PS-Simulink Converter27/1 -> Mux4/7
  PS-Simulink Converter15/1 -> Mux1/7
  PS-Simulink Converter16/1 -> Mux2/4
  Demux/7 -> Simulink-PS Converter6/1
  Demux/3 -> Simulink-PS Converter2/1
  PS-Simulink Converter28/1 -> Mux4/1
  PS-Simulink Converter13/1 -> Mux1/5
  PS-Simulink Converter9/1 -> Mux1/1
  Demux/6 -> Simulink-PS Converter5/1
  PS-Simulink Converter1/1 -> Mux2/3
  Demux/5 -> Simulink-PS Converter4/1
  PS-Simulink Converter24/1 -> Mux4/4
  Demux/4 -> Simulink-PS Converter3/1
  Mux4/1 -> qdotdot_real [rad/s2]/1
  Demux1/1 -> Simulink-PS Converter7/1
  Demux1/2 -> Simulink-PS Converter8/1
  Demux1/3 -> Simulink-PS Converter9/1
  Demux1/4 -> Simulink-PS Converter11/1
  Demux1/5 -> Simulink-PS Converter10/1
  Demux1/6 -> Simulink-PS Converter12/1
  tao0/1 -> Demux1/1
  PS-Simulink Converter17/1 -> Coordinate Transformation Conversion1/1
  PS-Simulink Converter34/1 -> Mux6/1
  PS-Simulink Converter35/1 -> Mux6/2
  PS-Simulink Converter36/1 -> Mux6/3
  Coordinate Transformation Conversion1/1 -> "world_Rotm_base "/1
  Mux6/1 -> world_position_base/1
  connections:
  Joint_6/LConn1 -- Link_5/RConn1
  6-DOF Joint/RConn8 -- PS-Simulink Converter16/LConn1
  6-DOF Joint/RConn5 -- PS-Simulink Converter1/LConn1
  Joint_4/LConn1 -- Link_3/RConn1
  Joint_3/LConn1 -- Link_2/RConn1
  Chaser_Spacecraft/LConn1 -- 6-DOF Joint/RConn1 -- Transform Sensor/RConn1
  Joint_6/RConn2 -- PS-Simulink Converter7/LConn1
  Link_5/LConn1 -- Joint_5/RConn1
  Joint_EE/RConn1 -- Link_EE/LConn1
  Joint_4/RConn3 -- PS-Simulink Converter12/LConn1
  Link_6/RConn1 -- Joint_7/LConn1
  Chaser_Spacecraft/RConn1 -- Joint_1/LConn1
  Joint_2/RConn4 -- PS-Simulink Converter22/LConn1
  Joint_6/RConn4 -- PS-Simulink Converter26/LConn1
  6-DOF Joint/RConn2 -- PS-Simulink Converter/LConn1
  PS-Simulink Converter31/LConn1 -- 6-DOF Joint/RConn7
  Joint_2/RConn2 -- PS-Simulink Converter3/LConn1
  Joint_2/RConn1 -- Link_2/LConn1
  Simulink-PS Converter1/RConn1 -- Joint_2/LConn2
  Joint_4/RConn2 -- PS-Simulink Converter5/LConn1
  6-DOF Joint/RConn3 -- PS-Simulink Converter18/LConn1
  PS-Simulink Converter30/LConn1 -- 6-DOF Joint/RConn4
  Joint_5/RConn4 -- PS-Simulink Converter25/LConn1
  Joint_1/RConn3 -- PS-Simulink Converter9/LConn1
  6-DOF Joint/RConn11 -- PS-Simulink Converter20/LConn1
  Joint_7/RConn2 -- PS-Simulink Converter8/LConn1
  Joint_4/RConn4 -- PS-Simulink Converter24/LConn1
  Joint_3/RConn1 -- Link_3/LConn1
  Solver Configuration/RConn1 -- Transform Sensor/LConn1 -- 6-DOF Joint/LConn1 -- World/RConn1 -- MechanismConfiguration/RConn1
  Simulink-PS Converter/RConn1 -- Joint_1/LConn2
  Simulink-PS Converter2/RConn1 -- Joint_3/LConn2
  Link_6/LConn1 -- Joint_6/RConn1
  Joint_3/RConn3 -- PS-Simulink Converter11/LConn1
  Joint_2/LConn1 -- Link_1/RConn1
  Simulink-PS Converter4/RConn1 -- Joint_5/LConn2
  Link_7/LConn1 -- Joint_7/RConn1
  Joint_1/RConn4 -- PS-Simulink Converter28/LConn1
  Joint_5/LConn1 -- Link_4/RConn1
  Joint_7/RConn4 -- PS-Simulink Converter27/LConn1
  Joint_3/RConn2 -- PS-Simulink Converter4/LConn1
  6-DOF Joint/RConn9 -- PS-Simulink Converter21/LConn1
  Joint_1/RConn2 -- PS-Simulink Converter2/LConn1
  Joint_6/RConn3 -- PS-Simulink Converter14/LConn1
  6-DOF Joint/RConn6 -- PS-Simulink Converter19/LConn1
  Joint_2/RConn3 -- PS-Simulink Converter10/LConn1
  Joint_7/RConn3 -- PS-Simulink Converter15/LConn1
  Joint_1/RConn1 -- Link_1/LConn1
  PS-Simulink Converter32/LConn1 -- 6-DOF Joint/RConn10
  Joint_3/RConn4 -- PS-Simulink Converter23/LConn1
  Joint_EE/LConn1 -- Link_7/RConn1
  Joint_6/LConn2 -- Simulink-PS Converter5/RConn1
  PS-Simulink Converter29/LConn1 -- 6-DOF Joint/RConn13
  Joint_5/RConn2 -- PS-Simulink Converter6/LConn1
  Simulink-PS Converter6/RConn1 -- Joint_7/LConn2
  Joint_4/RConn1 -- Link_4/LConn1
  Joint_5/RConn3 -- PS-Simulink Converter13/LConn1
  Simulink-PS Converter3/RConn1 -- Joint_4/LConn2
  Simulink-PS Converter7/RConn1 -- 6-DOF Joint/LConn5
  Simulink-PS Converter8/RConn1 -- 6-DOF Joint/LConn6
  Simulink-PS Converter9/RConn1 -- 6-DOF Joint/LConn7
  Simulink-PS Converter11/RConn1 -- 6-DOF Joint/LConn2
  Simulink-PS Converter10/RConn1 -- 6-DOF Joint/LConn3
  Simulink-PS Converter12/RConn1 -- 6-DOF Joint/LConn4
  PS-Simulink Converter33/LConn1 -- 6-DOF Joint/RConn12
  PS-Simulink Converter17/LConn1 -- Transform Sensor/RConn2
  Transform Sensor/RConn3 -- PS-Simulink Converter34/LConn1
  Transform Sensor/RConn4 -- PS-Simulink Converter35/LConn1
  Transform Sensor/RConn5 -- PS-Simulink Converter36/LConn1

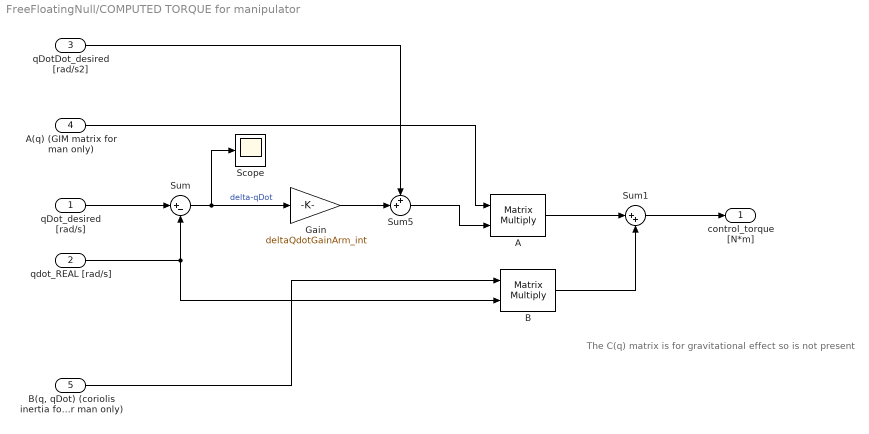
== system FreeFloatingNull/COMPUTED TORQUE for manipulator ==
  note: The C(q) matrix is for gravitational effect so is not present
  qDot_desired [rad/s] : Inport
  qdot_REAL [rad/s] : Inport  Port=2
  qDotDot_desired [rad/s2] : Inport  Port=3
  A(q) (GIM matrix for man only) : Inport  Port=4
  "B(q, qDot) (coriolis inertia for man only)" : Inport  Port=5
  A : Product  Multiplication=Matrix(*)
  B : Product  Multiplication=Matrix(*)
  Gain : Gain  Gain=deltaQdotGainArm_int
  Scope : Scope
  Sum : Sum  Inputs=|+-
  Sum1 : Sum  Inputs=|++
  Sum5 : Sum  Inputs=++|
  control_torque [N*m] : Outport
  wires:
  qDot_desired [rad/s]/1 -> Sum/1
  qDotDot_desired [rad/s2]/1 -> Sum5/1
  Sum/1 -> Scope/1, Gain/1  "delta-qDot"
  A(q) (GIM matrix for man only)/1 -> A/1
  A/1 -> Sum1/1
  Sum5/1 -> A/2
  "B(q, qDot) (coriolis inertia for man only)"/1 -> B/1
  Sum1/1 -> control_torque [N*m]/1
  qdot_REAL [rad/s]/1 -> B/2, Sum/2
  B/1 -> Sum1/2
  Gain/1 -> Sum5/2

== system FreeFloatingNull/Desired Position Linear [m]  ==
  Bus Creator : BusCreator  Tag=Bus Creator  Inputs=3
  FromWs : FromWorkspace  Tag=STV FromWs  VariableName=tuvar  SampleTime=0
      SigBuilderData=|
      | common.afterFinalStr = 'Extrapolate'
      | common.sampleTime = 0
      | dataSet(1).timeRange = [0 30]
      | dataSet(1).name = 'Position'
      | dataSet(2).timeRange = [0 30]
      | dataSet(2).name = 'Position1'
      | sbobj.Groups(1).Name = 'Position'
      | sbobj.Groups(1).Signals(1).Name = 'Position x'
      | sbobj.Groups(1).Signals(1).XData = [0 0.15075 0.3015 0.45226 0.60301 0.75376 0.90451 1.0553 1.206 1.3568 1.5075 1.6583 1.809 1.9598 2.1105 2.2613 2.412 2.5628 2.7135 2.8643 3.015 3.1658 3.3165 3.4673 3.618 3.7688 3.9196 4.0703 4.2211 4.3718 4.5226 4.6733 4.8241 4.9748 5.1256 5.2763 5.4271 5.5778 5.7286 5.8793 6.0301 6.1808 6.3316 6.4823 6.6331 6.7838 6.9346 7.0853 7.2361 7.3869 7.5376 7.6884 7.8391 7.9899 8.1406 8.2914 8.4421 8.5929 8.7436 8.8944 9.0451 9.1959 9.3466 9.4974 9.6481 9.7989 9.9496 10.1 10.251 10.402 10.553 10.703 10.854 11.005 11.156 11.306 11.457 11.608 11.759 11.909 12.06 12.211 12.362 12.512 12.663 12.814 12.965 13.115 13.266 13.417 13.568 13.718 13.869 14.02 14.171 14.321 14.472 14.623 14.774 14.924 15.075 15.226 15.377 15.527 15.678 15.829 15.98 16.13 16.281 16.432 16.583 16.733 16.884 17.035 17.186 17.336 17.487 17.638 17.789 17.939 18.09 18.241 18.392 18.543 18.693 18.844 18.995 19.146 19.296 19.447 19.598 19.749 19.899 20.05 20.201 20.352 20.502 20.653 20.804 20.955 21.105 21.256 21.407 21.558 21.708 21.859 22.01 22.161 22.311 22.462 22.613 22.764 22.914 23.065 23.216 23.367 23.517 23.668 23.819 23.97 24.12 24.271 24.422 24.573 24.723 24.874 25.025 25.176 25.326 25.477 25.628 25.779 25.929 26.08 26.231 26.382 26.532 26.683 26.834 26.985 27.135 27.286 27.437 27.588 27.738 27.889 28.04 28.191 28.341 28.492 28.643 28.794 28.944 29.095 29.246 29.397 29.547 29.698 29.849 30]
      | sbobj.Groups(1).Signals(1).YData = [4.1497 4.1496 4.1494 4.149 4.1484 4.1474 4.1461 4.1445 4.1427 4.1405 4.1382 4.1356 4.1328 4.1298 4.1268 4.1236 4.1203 4.117 4.1136 4.1102 4.1067 4.1033 4.0999 4.0964 4.093 4.0896 4.0862 4.0828 4.0794 4.076 4.0726 4.0692 4.0657 4.0622 4.0586 4.055 4.0513 4.0476 4.0438 4.0399 4.0359 4.0318 4.0277 4.0235 4.0192 4.0148 4.0104 4.0058 4.0012 3.9966 3.9918 3.987 3.9822 3.9773 3.9723 3.9674 3.9623 3.9573 3.9522 3.9471 3.9419 3.9368 3.9316 3.9265 3.9213 3.9161 3.9109 3.9056 3.9004 3.8951 3.8899 3.8846 3.8793 3.8739 3.8686 3.8632 3.8578 3.8523 3.8468 3.8413 3.8357 3.83 3.8243 3.8186 3.8128 3.8069 3.801 3.795 3.7889 3.7828 3.7766 3.7704 3.7641 3.7578 3.7513 3.7449 3.7384 3.7318 3.7252 3.7186 3.7119 3.7052 3.6984 3.6917 3.6849 3.678 3.6712 3.6644 3.6575 3.6506 3.6438 3.6369 3.63 3.6231 3.6163 3.6094 3.6025 3.5956 3.5887 3.5818 3.5749 3.5679 3.561 3.554 3.547 3.54 3.533 3.5259 3.5188 3.5116 3.5044 3.4972 3.4899 3.4825 3.4751 3.4676 3.4601 3.4525 3.4449 3.4371 3.4294 3.4216 3.4137 3.4058 3.3978 3.3898 3.3818 3.3737 3.3656 3.3575 3.3494 3.3412 3.3331 3.325 3.3169 3.3088 3.3007 3.2927 3.2847 3.2767 3.2687 3.2608 3.253 3.2451 3.2373 3.2295 3.2217 3.2139 3.2061 3.1983 3.1905 3.1826 3.1747 3.1668 3.1587 3.1506 3.1424 3.1341 3.1258 3.1173 3.1087 3.1 3.0912 3.0824 3.0736 3.0647 3.0559 3.0471 3.0385 3.0301 3.022 3.0143 3.0071 3.0004 2.9944 2.9892 2.9849 2.9817 2.9797 2.979]
      | sbobj.Groups(1).Signals(2).Name = 'Position y'
      | sbobj.Groups(1).Signals(2).XData = [0 0.15075 0.3015 0.45226 0.60301 0.75376 0.90451 1.0553 1.206 1.3568 1.5075 1.6583 1.809 1.9598 2.1105 2.2613 2.412 2.5628 2.7135 2.8643 3.015 3.1658 3.3165 3.4673 3.618 3.7688 3.9196 4.0703 4.2211 4.3718 4.5226 4.6733 4.8241 4.9748 5.1256 5.2763 5.4271 5.5778 5.7286 5.8793 6.0301 6.1808 6.3316 6.4823 6.6331 6.7838 6.9346 7.0853 7.2361 7.3869 7.5376 7.6884 7.8391 7.9899 8.1406 8.2914 8.4421 8.5929 8.7436 8.8944 9.0451 9.1959 9.3466 9.4974 9.6481 9.7989 9.9496 10.1 10.251 10.402 10.553 10.703 10.854 11.005 11.156 11.306 11.457 11.608 11.759 11.909 12.06 12.211 12.362 12.512 12.663 12.814 12.965 13.115 13.266 13.417 13.568 13.718 13.869 14.02 14.171 14.321 14.472 14.623 14.774 14.924 15.075 15.226 15.377 15.527 15.678 15.829 15.98 16.13 16.281 16.432 16.583 16.733 16.884 17.035 17.186 17.336 17.487 17.638 17.789 17.939 18.09 18.241 18.392 18.543 18.693 18.844 18.995 19.146 19.296 19.447 19.598 19.749 19.899 20.05 20.201 20.352 20.502 20.653 20.804 20.955 21.105 21.256 21.407 21.558 21.708 21.859 22.01 22.161 22.311 22.462 22.613 22.764 22.914 23.065 23.216 23.367 23.517 23.668 23.819 23.97 24.12 24.271 24.422 24.573 24.723 24.874 25.025 25.176 25.326 25.477 25.628 25.779 25.929 26.08 26.231 26.382 26.532 26.683 26.834 26.985 27.135 27.286 27.437 27.588 27.738 27.889 28.04 28.191 28.341 28.492 28.643 28.794 28.944 29.095 29.246 29.397 29.547 29.698 29.849 30]
      | sbobj.Groups(1).Signals(2).YData = [0.16804 0.16819 0.16861 0.16923 0.17001 0.17093 0.17195 0.17305 0.1742 0.17541 0.17666 0.17793 0.17923 0.18054 0.18188 0.18322 0.18458 0.18595 0.18732 0.1887 0.19008 0.19147 0.19286 0.19425 0.19564 0.19703 0.19842 0.19981 0.2012 0.20259 0.20397 0.20535 0.20673 0.2081 0.20948 0.21085 0.21222 0.21359 0.21496 0.21632 0.21769 0.21906 0.22044 0.22181 0.22319 0.22458 0.22597 0.22738 0.22879 0.23021 0.23164 0.23309 0.23455 0.23602 0.23751 0.23902 0.24054 0.24207 0.24363 0.2452 0.24679 0.24839 0.25002 0.25166 0.25331 0.25498 0.25667 0.25837 0.26008 0.2618 0.26354 0.26528 0.26703 0.26879 0.27056 0.27233 0.27411 0.27589 0.27767 0.27945 0.28123 0.283 0.28478 0.28655 0.28832 0.29008 0.29184 0.2936 0.29535 0.2971 0.29884 0.30058 0.30231 0.30404 0.30577 0.30749 0.30922 0.31095 0.31268 0.31441 0.31614 0.31789 0.31963 0.32139 0.32316 0.32494 0.32673 0.32854 0.33036 0.3322 0.33405 0.33592 0.33782 0.33973 0.34166 0.34361 0.34558 0.34758 0.34959 0.35162 0.35367 0.35574 0.35782 0.35992 0.36204 0.36416 0.3663 0.36845 0.3706 0.37276 0.37493 0.37709 0.37926 0.38142 0.38358 0.38573 0.38788 0.39002 0.39214 0.39426 0.39636 0.39845 0.40052 0.40259 0.40464 0.40667 0.4087 0.41071 0.41272 0.41471 0.41671 0.4187 0.42069 0.42268 0.42468 0.42668 0.4287 0.43074 0.43279 0.43487 0.43697 0.43911 0.44128 0.44348 0.44572 0.44801 0.45033 0.4527 0.45511 0.45757 0.46008 0.46262 0.46521 0.46784 0.47051 0.47321 0.47593 0.47868 0.48145 0.48422 0.48701 0.48978 0.49255 0.49529 0.49801 0.50068 0.5033 0.50586 0.50835 0.51074 0.51304 0.51521 0.51725 0.51912 0.52082 0.5223 0.52353 0.52447 0.52508 0.52529]
      | sbobj.Groups(1).Signals(3).Name = 'Position z'
      | sbobj.Groups(1).Signals(3).XData = [0 0.15075 0.3015 0.45226 0.60301 0.75376 0.90451 1.0553 1.206 1.3568 1.5075 1.6583 1.809 1.9598 2.1105 2.2613 2.412 2.5628 2.7135 2.8643 3.015 3.1658 3.3165 3.4673 3.618 3.7688 3.9196 4.0703 4.2211 4.3718 4.5226 4.6733 4.8241 4.9748 5.1256 5.2763 5.4271 5.5778 5.7286 5.8793 6.0301 6.1808 6.3316 6.4823 6.6331 6.7838 6.9346 7.0853 7.2361 7.3869 7.5376 7.6884 7.8391 7.9899 8.1406 8.2914 8.4421 8.5929 8.7436 8.8944 9.0451 9.1959 9.3466 9.4974 9.6481 9.7989 9.9496 10.1 10.251 10.402 10.553 10.703 10.854 11.005 11.156 11.306 11.457 11.608 11.759 11.909 12.06 12.211 12.362 12.512 12.663 12.814 12.965 13.115 13.266 13.417 13.568 13.718 13.869 14.02 14.171 14.321 14.472 14.623 14.774 14.924 15.075 15.226 15.377 15.527 15.678 15.829 15.98 16.13 16.281 16.432 16.583 16.733 16.884 17.035 17.186 17.336 17.487 17.638 17.789 17.939 18.09 18.241 18.392 18.543 18.693 18.844 18.995 19.146 19.296 19.447 19.598 19.749 19.899 20.05 20.201 20.352 20.502 20.653 20.804 20.955 21.105 21.256 21.407 21.558 21.708 21.859 22.01 22.161 22.311 22.462 22.613 22.764 22.914 23.065 23.216 23.367 23.517 23.668 23.819 23.97 24.12 24.271 24.422 24.573 24.723 24.874 25.025 25.176 25.326 25.477 25.628 25.779 25.929 26.08 26.231 26.382 26.532 26.683 26.834 26.985 27.135 27.286 27.437 27.588 27.738 27.889 28.04 28.191 28.341 28.492 28.643 28.794 28.944 29.095 29.246 29.397 29.547 29.698 29.849 30]
      | sbobj.Groups(1).Signals(3).YData = [1.735 1.7355 1.737 1.7396 1.7435 1.7485 1.7547 1.7619 1.7701 1.7791 1.7889 1.7992 1.81 1.8211 1.8325 1.844 1.8557 1.8673 1.8789 1.8904 1.9017 1.9129 1.924 1.9348 1.9455 1.9559 1.9662 1.9764 1.9863 1.9962 2.0059 2.0155 2.0251 2.0346 2.044 2.0535 2.0629 2.0723 2.0817 2.0912 2.1007 2.1102 2.1198 2.1294 2.1391 2.1488 2.1585 2.1682 2.178 2.1878 2.1976 2.2074 2.2171 2.2269 2.2366 2.2463 2.2559 2.2655 2.275 2.2845 2.2939 2.3032 2.3124 2.3215 2.3306 2.3395 2.3484 2.3572 2.3659 2.3746 2.3831 2.3916 2.4 2.4083 2.4166 2.4248 2.4329 2.441 2.4491 2.4571 2.4651 2.4731 2.481 2.4889 2.4968 2.5047 2.5126 2.5204 2.5283 2.5361 2.5439 2.5518 2.5596 2.5674 2.5751 2.5829 2.5906 2.5983 2.606 2.6137 2.6213 2.6289 2.6364 2.6439 2.6513 2.6587 2.666 2.6733 2.6804 2.6876 2.6946 2.7016 2.7085 2.7153 2.722 2.7287 2.7353 2.7418 2.7483 2.7546 2.7609 2.7672 2.7733 2.7794 2.7855 2.7915 2.7974 2.8033 2.8091 2.815 2.8207 2.8265 2.8322 2.8379 2.8435 2.8492 2.8548 2.8604 2.866 2.8715 2.8771 2.8826 2.8881 2.8936 2.899 2.9045 2.9099 2.9152 2.9206 2.9258 2.9311 2.9362 2.9414 2.9464 2.9514 2.9563 2.9611 2.9659 2.9705 2.9751 2.9796 2.984 2.9883 2.9925 2.9966 3.0006 3.0045 3.0084 3.0122 3.0159 3.0195 3.0231 3.0266 3.0301 3.0336 3.037 3.0404 3.0438 3.0472 3.0506 3.054 3.0573 3.0607 3.0641 3.0674 3.0707 3.0739 3.0771 3.0802 3.0832 3.086 3.0887 3.0911 3.0934 3.0953 3.097 3.0983 3.0992 3.0998 3.1]
      | sbobj.Groups(1).TimeRange = [0 30]
      | sbobj.Groups(2).Name = 'Position1'
      | sbobj.Groups(2).Signals(1).Name = 'Position x'
      | sbobj.Groups(2).Signals(1).XData = [0 0.15075 0.3015 0.45226 0.60301 0.75376 0.90451 1.0553 1.206 1.3568 1.5075 1.6583 1.809 1.9598 2.1105 2.2613 2.412 2.5628 2.7135 2.8643 3.015 3.1658 3.3165 3.4673 3.618 3.7688 3.9196 4.0703 4.2211 4.3718 4.5226 4.6733 4.8241 4.9748 5.1256 5.2763 5.4271 5.5778 5.7286 5.8793 6.0301 6.1808 6.3316 6.4823 6.6331 6.7838 6.9346 7.0853 7.2361 7.3869 7.5376 7.6884 7.8391 7.9899 8.1406 8.2914 8.4421 8.5929 8.7436 8.8944 9.0451 9.1959 9.3466 9.4974 9.6481 9.7989 9.9496 10.1 10.251 10.402 10.553 10.703 10.854 11.005 11.156 11.306 11.457 11.608 11.759 11.909 12.06 12.211 12.362 12.512 12.663 12.814 12.965 13.115 13.266 13.417 13.568 13.718 13.869 14.02 14.171 14.321 14.472 14.623 14.774 14.924 15.075 15.226 15.377 15.527 15.678 15.829 15.98 16.13 16.281 16.432 16.583 16.733 16.884 17.035 17.186 17.336 17.487 17.638 17.789 17.939 18.09 18.241 18.392 18.543 18.693 18.844 18.995 19.146 19.296 19.447 19.598 19.749 19.899 20.05 20.201 20.352 20.502 20.653 20.804 20.955 21.105 21.256 21.407 21.558 21.708 21.859 22.01 22.161 22.311 22.462 22.613 22.764 22.914 23.065 23.216 23.367 23.517 23.668 23.819 23.97 24.12 24.271 24.422 24.573 24.723 24.874 25.025 25.176 25.326 25.477 25.628 25.779 25.929 26.08 26.231 26.382 26.532 26.683 26.834 26.985 27.135 27.286 27.437 27.588 27.738 27.889 28.04 28.191 28.341 28.492 28.643 28.794 28.944 29.095 29.246 29.397 29.547 29.698 29.849 30]
      | sbobj.Groups(2).Signals(1).YData = [4.1497 4.1496 4.1494 4.149 4.1484 4.1474 4.1461 4.1445 4.1427 4.1405 4.1382 4.1356 4.1328 4.1298 4.1268 4.1236 4.1203 4.117 4.1136 4.1102 4.1067 4.1033 4.0999 4.0964 4.093 4.0896 4.0862 4.0828 4.0794 4.076 4.0726 4.0692 4.0657 4.0622 4.0586 4.055 4.0513 4.0476 4.0438 4.0399 4.0359 4.0318 4.0277 4.0235 4.0192 4.0148 4.0104 4.0058 4.0012 3.9966 3.9918 3.987 3.9822 3.9773 3.9723 3.9674 3.9623 3.9573 3.9522 3.9471 3.9419 3.9368 3.9316 3.9265 3.9213 3.9161 3.9109 3.9056 3.9004 3.8951 3.8899 3.8846 3.8793 3.8739 3.8686 3.8632 3.8578 3.8523 3.8468 3.8413 3.8357 3.83 3.8243 3.8186 3.8128 3.8069 3.801 3.795 3.7889 3.7828 3.7766 3.7704 3.7641 3.7578 3.7513 3.7449 3.7384 3.7318 3.7252 3.7186 3.7119 3.7052 3.6984 3.6917 3.6849 3.678 3.6712 3.6644 3.6575 3.6506 3.6438 3.6369 3.63 3.6231 3.6163 3.6094 3.6025 3.5956 3.5887 3.5818 3.5749 3.5679 3.561 3.554 3.547 3.54 3.533 3.5259 3.5188 3.5116 3.5044 3.4972 3.4899 3.4825 3.4751 3.4676 3.4601 3.4525 3.4449 3.4371 3.4294 3.4216 3.4137 3.4058 3.3978 3.3898 3.3818 3.3737 3.3656 3.3575 3.3494 3.3412 3.3331 3.325 3.3169 3.3088 3.3007 3.2927 3.2847 3.2767 3.2687 3.2608 3.253 3.2451 3.2373 3.2295 3.2217 3.2139 3.2061 3.1983 3.1905 3.1826 3.1747 3.1668 3.1587 3.1506 3.1424 3.1341 3.1258 3.1173 3.1087 3.1 3.0912 3.0824 3.0736 3.0647 3.0559 3.0471 3.0385 3.0301 3.022 3.0143 3.0071 3.0004 2.9944 2.9892 2.9849 2.9817 2.9797 2.979]
      | sbobj.Groups(2).Signals(2).Name = 'Position y'
      | sbobj.Groups(2).Signals(2).XData = [0 0.15075 0.3015 0.45226 0.60301 0.75376 0.90451 1.0553 1.206 1.3568 1.5075 1.6583 1.809 1.9598 2.1105 2.2613 2.412 2.5628 2.7135 2.8643 3.015 3.1658 3.3165 3.4673 3.618 3.7688 3.9196 4.0703 4.2211 4.3718 4.5226 4.6733 4.8241 4.9748 5.1256 5.2763 5.4271 5.5778 5.7286 5.8793 6.0301 6.1808 6.3316 6.4823 6.6331 6.7838 6.9346 7.0853 7.2361 7.3869 7.5376 7.6884 7.8391 7.9899 8.1406 8.2914 8.4421 8.5929 8.7436 8.8944 9.0451 9.1959 9.3466 9.4974 9.6481 9.7989 9.9496 10.1 10.251 10.402 10.553 10.703 10.854 11.005 11.156 11.306 11.457 11.608 11.759 11.909 12.06 12.211 12.362 12.512 12.663 12.814 12.965 13.115 13.266 13.417 13.568 13.718 13.869 14.02 14.171 14.321 14.472 14.623 14.774 14.924 15.075 15.226 15.377 15.527 15.678 15.829 15.98 16.13 16.281 16.432 16.583 16.733 16.884 17.035 17.186 17.336 17.487 17.638 17.789 17.939 18.09 18.241 18.392 18.543 18.693 18.844 18.995 19.146 19.296 19.447 19.598 19.749 19.899 20.05 20.201 20.352 20.502 20.653 20.804 20.955 21.105 21.256 21.407 21.558 21.708 21.859 22.01 22.161 22.311 22.462 22.613 22.764 22.914 23.065 23.216 23.367 23.517 23.668 23.819 23.97 24.12 24.271 24.422 24.573 24.723 24.874 25.025 25.176 25.326 25.477 25.628 25.779 25.929 26.08 26.231 26.382 26.532 26.683 26.834 26.985 27.135 27.286 27.437 27.588 27.738 27.889 28.04 28.191 28.341 28.492 28.643 28.794 28.944 29.095 29.246 29.397 29.547 29.698 29.849 30]
      | sbobj.Groups(2).Signals(2).YData = [0.16804 0.16819 0.16861 0.16923 0.17001 0.17093 0.17195 0.17305 0.1742 0.17541 0.17666 0.17793 0.17923 0.18054 0.18188 0.18322 0.18458 0.18595 0.18732 0.1887 0.19008 0.19147 0.19286 0.19425 0.19564 0.19703 0.19842 0.19981 0.2012 0.20259 0.20397 0.20535 0.20673 0.2081 0.20948 0.21085 0.21222 0.21359 0.21496 0.21632 0.21769 0.21906 0.22044 0.22181 0.22319 0.22458 0.22597 0.22738 0.22879 0.23021 0.23164 0.23309 0.23455 0.23602 0.23751 0.23902 0.24054 0.24207 0.24363 0.2452 0.24679 0.24839 0.25002 0.25166 0.25331 0.25498 0.25667 0.25837 0.26008 0.2618 0.26354 0.26528 0.26703 0.26879 0.27056 0.27233 0.27411 0.27589 0.27767 0.27945 0.28123 0.283 0.28478 0.28655 0.28832 0.29008 0.29184 0.2936 0.29535 0.2971 0.29884 0.30058 0.30231 0.30404 0.30577 0.30749 0.30922 0.31095 0.31268 0.31441 0.31614 0.31789 0.31963 0.32139 0.32316 0.32494 0.32673 0.32854 0.33036 0.3322 0.33405 0.33592 0.33782 0.33973 0.34166 0.34361 0.34558 0.34758 0.34959 0.35162 0.35367 0.35574 0.35782 0.35992 0.36204 0.36416 0.3663 0.36845 0.3706 0.37276 0.37493 0.37709 0.37926 0.38142 0.38358 0.38573 0.38788 0.39002 0.39214 0.39426 0.39636 0.39845 0.40052 0.40259 0.40464 0.40667 0.4087 0.41071 0.41272 0.41471 0.41671 0.4187 0.42069 0.42268 0.42468 0.42668 0.4287 0.43074 0.43279 0.43487 0.43697 0.43911 0.44128 0.44348 0.44572 0.44801 0.45033 0.4527 0.45511 0.45757 0.46008 0.46262 0.46521 0.46784 0.47051 0.47321 0.47593 0.47868 0.48145 0.48422 0.48701 0.48978 0.49255 0.49529 0.49801 0.50068 0.5033 0.50586 0.50835 0.51074 0.51304 0.51521 0.51725 0.51912 0.52082 0.5223 0.52353 0.52447 0.52508 0.52529]
      | sbobj.Groups(2).Signals(3).Name = 'Position z'
      | sbobj.Groups(2).Signals(3).XData = [0 0.15075 0.3015 0.45226 0.60301 0.75376 0.90451 1.0553 1.206 1.3568 1.5075 1.6583 1.809 1.9598 2.1105 2.2613 2.412 2.5628 2.7135 2.8643 3.015 3.1658 3.3165 3.4673 3.618 3.7688 3.9196 4.0703 4.2211 4.3718 4.5226 4.6733 4.8241 4.9748 5.1256 5.2763 5.4271 5.5778 5.7286 5.8793 6.0301 6.1808 6.3316 6.4823 6.6331 6.7838 6.9346 7.0853 7.2361 7.3869 7.5376 7.6884 7.8391 7.9899 8.1406 8.2914 8.4421 8.5929 8.7436 8.8944 9.0451 9.1959 9.3466 9.4974 9.6481 9.7989 9.9496 10.1 10.251 10.402 10.553 10.703 10.854 11.005 11.156 11.306 11.457 11.608 11.759 11.909 12.06 12.211 12.362 12.512 12.663 12.814 12.965 13.115 13.266 13.417 13.568 13.718 13.869 14.02 14.171 14.321 14.472 14.623 14.774 14.924 15.075 15.226 15.377 15.527 15.678 15.829 15.98 16.13 16.281 16.432 16.583 16.733 16.884 17.035 17.186 17.336 17.487 17.638 17.789 17.939 18.09 18.241 18.392 18.543 18.693 18.844 18.995 19.146 19.296 19.447 19.598 19.749 19.899 20.05 20.201 20.352 20.502 20.653 20.804 20.955 21.105 21.256 21.407 21.558 21.708 21.859 22.01 22.161 22.311 22.462 22.613 22.764 22.914 23.065 23.216 23.367 23.517 23.668 23.819 23.97 24.12 24.271 24.422 24.573 24.723 24.874 25.025 25.176 25.326 25.477 25.628 25.779 25.929 26.08 26.231 26.382 26.532 26.683 26.834 26.985 27.135 27.286 27.437 27.588 27.738 27.889 28.04 28.191 28.341 28.492 28.643 28.794 28.944 29.095 29.246 29.397 29.547 29.698 29.849 30]
      | sbobj.Groups(2).Signals(3).YData = [1.735 1.7355 1.737 1.7396 1.7435 1.7485 1.7547 1.7619 1.7701 1.7791 1.7889 1.7992 1.81 1.8211 1.8325 1.844 1.8557 1.8673 1.8789 1.8904 1.9017 1.9129 1.924 1.9348 1.9455 1.9559 1.9662 1.9764 1.9863 1.9962 2.0059 2.0155 2.0251 2.0346 2.044 2.0535 2.0629 2.0723 2.0817 2.0912 2.1007 2.1102 2.1198 2.1294 2.1391 2.1488 2.1585 2.1682 2.178 2.1878 2.1976 2.2074 2.2171 2.2269 2.2366 2.2463 2.2559 2.2655 2.275 2.2845 2.2939 2.3032 2.3124 2.3215 2.3306 2.3395 2.3484 2.3572 2.3659 2.3746 2.3831 2.3916 2.4 2.4083 2.4166 2.4248 2.4329 2.441 2.4491 2.4571 2.4651 2.4731 2.481 2.4889 2.4968 2.5047 2.5126 2.5204 2.5283 2.5361 2.5439 2.5518 2.5596 2.5674 2.5751 2.5829 2.5906 2.5983 2.606 2.6137 2.6213 2.6289 2.6364 2.6439 2.6513 2.6587 2.666 2.6733 2.6804 2.6876 2.6946 2.7016 2.7085 2.7153 2.722 2.7287 2.7353 2.7418 2.7483 2.7546 2.7609 2.7672 2.7733 2.7794 2.7855 2.7915 2.7974 2.8033 2.8091 2.815 2.8207 2.8265 2.8322 2.8379 2.8435 2.8492 2.8548 2.8604 2.866 2.8715 2.8771 2.8826 2.8881 2.8936 2.899 2.9045 2.9099 2.9152 2.9206 2.9258 2.9311 2.9362 2.9414 2.9464 2.9514 2.9563 2.9611 2.9659 2.9705 2.9751 2.9796 2.984 2.9883 2.9925 2.9966 3.0006 3.0045 3.0084 3.0122 3.0159 3.0195 3.0231 3.0266 3.0301 3.0336 3.037 3.0404 3.0438 3.0472 3.0506 3.054 3.0573 3.0607 3.0641 3.0674 3.0707 3.0739 3.0771 3.0802 3.0832 3.086 3.0887 3.0911 3.0934 3.0953 3.097 3.0983 3.0992 3.0998 3.1]
      | sbobj.Groups(2).TimeRange = [0 30]
  Subsystem : Subsystem
  Bus : Outport
  wires:
  FromWs/1 -> Subsystem/1(In1)
  Bus Creator/1 -> Bus/1
  Subsystem/1(Position x) -> Bus Creator/1  "Position x"
  Subsystem/2(Position y) -> Bus Creator/2  "Position y"
  Subsystem/3(Position z) -> Bus Creator/3  "Position z"

== system FreeFloatingNull/Desired Position angular [rad]1 ==
  Bus Creator : BusCreator  Tag=Bus Creator  Inputs=3
  FromWs : FromWorkspace  Tag=STV FromWs  VariableName=tuvar  SampleTime=0
      SigBuilderData=|
      | common.afterFinalStr = 'Extrapolate'
      | common.sampleTime = 0
      | dataSet(1).timeRange = [0 30]
      | dataSet(1).name = 'Position'
      | dataSet(2).timeRange = [0 30]
      | dataSet(2).name = 'Position1'
      | sbobj.Groups(1).Name = 'Position'
      | sbobj.Groups(1).Signals(1).Name = 'Position Angular x'
      | sbobj.Groups(1).Signals(1).XData = [0 0.15075 0.3015 0.45226 0.60301 0.75376 0.90451 1.0553 1.206 1.3568 1.5075 1.6583 1.809 1.9598 2.1105 2.2613 2.412 2.5628 2.7135 2.8643 3.015 3.1658 3.3165 3.4673 3.618 3.7688 3.9196 4.0703 4.2211 4.3718 4.5226 4.6733 4.8241 4.9748 5.1256 5.2763 5.4271 5.5778 5.7286 5.8793 6.0301 6.1808 6.3316 6.4823 6.6331 6.7838 6.9346 7.0853 7.2361 7.3869 7.5376 7.6884 7.8391 7.9899 8.1406 8.2914 8.4421 8.5929 8.7436 8.8944 9.0451 9.1959 9.3466 9.4974 9.6481 9.7989 9.9496 10.1 10.251 10.402 10.553 10.703 10.854 11.005 11.156 11.306 11.457 11.608 11.759 11.909 12.06 12.211 12.362 12.512 12.663 12.814 12.965 13.115 13.266 13.417 13.568 13.718 13.869 14.02 14.171 14.321 14.472 14.623 14.774 14.924 15.075 15.226 15.377 15.527 15.678 15.829 15.98 16.13 16.281 16.432 16.583 16.733 16.884 17.035 17.186 17.336 17.487 17.638 17.789 17.939 18.09 18.241 18.392 18.543 18.693 18.844 18.995 19.146 19.296 19.447 19.598 19.749 19.899 20.05 20.201 20.352 20.502 20.653 20.804 20.955 21.105 21.256 21.407 21.558 21.708 21.859 22.01 22.161 22.311 22.462 22.613 22.764 22.914 23.065 23.216 23.367 23.517 23.668 23.819 23.97 24.12 24.271 24.422 24.573 24.723 24.874 25.025 25.176 25.326 25.477 25.628 25.779 25.929 26.08 26.231 26.382 26.532 26.683 26.834 26.985 27.135 27.286 27.437 27.588 27.738 27.889 28.04 28.191 28.341 28.492 28.643 28.794 28.944 29.095 29.246 29.397 29.547 29.698 29.849 30]
      | sbobj.Groups(1).Signals(1).YData = [-1.2662 -2.371 -2.4879 -2.5537 -2.6023 -2.6406 -2.6717 -2.6974 -2.7189 -2.7372 -2.7527 -2.7661 -2.7777 -2.7877 -2.7963 -2.8039 -2.8104 -2.8161 -2.821 -2.8252 -2.8289 -2.832 -2.8346 -2.8369 -2.8388 -2.8404 -2.8417 -2.8429 -2.8438 -2.8446 -2.8453 -2.8459 -2.8464 -2.8469 -2.8474 -2.8479 -2.8484 -2.8489 -2.8495 -2.85 -2.8507 -2.8513 -2.852 -2.8528 -2.8536 -2.8544 -2.8552 -2.856 -2.8569 -2.8577 -2.8586 -2.8594 -2.8602 -2.861 -2.8617 -2.8624 -2.863 -2.8636 -2.8641 -2.8646 -2.865 -2.8654 -2.8656 -2.8659 -2.866 -2.8662 -2.8662 -2.8662 -2.8662 -2.8661 -2.866 -2.8659 -2.8657 -2.8655 -2.8653 -2.8651 -2.8649 -2.8647 -2.8645 -2.8643 -2.8641 -2.8639 -2.8638 -2.8637 -2.8636 -2.8635 -2.8635 -2.8635 -2.8635 -2.8636 -2.8637 -2.8638 -2.864 -2.8641 -2.8643 -2.8646 -2.8648 -2.865 -2.8653 -2.8655 -2.8658 -2.866 -2.8662 -2.8664 -2.8666 -2.8668 -2.8669 -2.867 -2.8671 -2.8672 -2.8672 -2.8672 -2.8671 -2.867 -2.8668 -2.8666 -2.8664 -2.8662 -2.8659 -2.8655 -2.8652 -2.8648 -2.8644 -2.864 -2.8635 -2.863 -2.8626 -2.8621 -2.8616 -2.8612 -2.8607 -2.8602 -2.8598 -2.8594 -2.859 -2.8586 -2.8582 -2.8579 -2.8576 -2.8573 -2.8571 -2.8568 -2.8566 -2.8565 -2.8563 -2.8562 -2.8561 -2.856 -2.8559 -2.8558 -2.8557 -2.8556 -2.8555 -2.8554 -2.8553 -2.8551 -2.8549 -2.8547 -2.8544 -2.8541 -2.8538 -2.8534 -2.853 -2.8525 -2.852 -2.8514 -2.8508 -2.8502 -2.8495 -2.8487 -2.8479 -2.8471 -2.8463 -2.8454 -2.8445 -2.8436 -2.8428 -2.8419 -2.841 -2.8401 -2.8393 -2.8384 -2.8376 -2.8368 -2.8361 -2.8354 -2.8347 -2.834 -2.8334 -2.8328 -2.8322 -2.8317 -2.8312 -2.8307 -2.8303 -2.8299 -2.8295 -2.8292 -2.8291 -2.8291]
      | sbobj.Groups(1).Signals(2).Name = 'Position Angular y'
      | sbobj.Groups(1).Signals(2).XData = [0 0.15075 0.3015 0.45226 0.60301 0.75376 0.90451 1.0553 1.206 1.3568 1.5075 1.6583 1.809 1.9598 2.1105 2.2613 2.412 2.5628 2.7135 2.8643 3.015 3.1658 3.3165 3.4673 3.618 3.7688 3.9196 4.0703 4.2211 4.3718 4.5226 4.6733 4.8241 4.9748 5.1256 5.2763 5.4271 5.5778 5.7286 5.8793 6.0301 6.1808 6.3316 6.4823 6.6331 6.7838 6.9346 7.0853 7.2361 7.3869 7.5376 7.6884 7.8391 7.9899 8.1406 8.2914 8.4421 8.5929 8.7436 8.8944 9.0451 9.1959 9.3466 9.4974 9.6481 9.7989 9.9496 10.1 10.251 10.402 10.553 10.703 10.854 11.005 11.156 11.306 11.457 11.608 11.759 11.909 12.06 12.211 12.362 12.512 12.663 12.814 12.965 13.115 13.266 13.417 13.568 13.718 13.869 14.02 14.171 14.321 14.472 14.623 14.774 14.924 15.075 15.226 15.377 15.527 15.678 15.829 15.98 16.13 16.281 16.432 16.583 16.733 16.884 17.035 17.186 17.336 17.487 17.638 17.789 17.939 18.09 18.241 18.392 18.543 18.693 18.844 18.995 19.146 19.296 19.447 19.598 19.749 19.899 20.05 20.201 20.352 20.502 20.653 20.804 20.955 21.105 21.256 21.407 21.558 21.708 21.859 22.01 22.161 22.311 22.462 22.613 22.764 22.914 23.065 23.216 23.367 23.517 23.668 23.819 23.97 24.12 24.271 24.422 24.573 24.723 24.874 25.025 25.176 25.326 25.477 25.628 25.779 25.929 26.08 26.231 26.382 26.532 26.683 26.834 26.985 27.135 27.286 27.437 27.588 27.738 27.889 28.04 28.191 28.341 28.492 28.643 28.794 28.944 29.095 29.246 29.397 29.547 29.698 29.849 30]
      | sbobj.Groups(1).Signals(2).YData = [-1.5708 -1.5706 -1.5699 -1.5687 -1.5669 -1.5646 -1.5618 -1.5584 -1.5546 -1.5504 -1.5458 -1.5409 -1.5358 -1.5305 -1.525 -1.5195 -1.5138 -1.5082 -1.5025 -1.4969 -1.4914 -1.4859 -1.4804 -1.4751 -1.4698 -1.4647 -1.4596 -1.4546 -1.4496 -1.4447 -1.4399 -1.4351 -1.4303 -1.4255 -1.4208 -1.416 -1.4113 -1.4065 -1.4017 -1.3969 -1.392 -1.3871 -1.3822 -1.3772 -1.3722 -1.3672 -1.3621 -1.3569 -1.3518 -1.3466 -1.3414 -1.3361 -1.3309 -1.3256 -1.3204 -1.3151 -1.3098 -1.3046 -1.2993 -1.2941 -1.2889 -1.2837 -1.2785 -1.2734 -1.2683 -1.2632 -1.2582 -1.2532 -1.2482 -1.2432 -1.2383 -1.2334 -1.2285 -1.2236 -1.2187 -1.2139 -1.2091 -1.2042 -1.1994 -1.1946 -1.1898 -1.185 -1.1801 -1.1753 -1.1704 -1.1655 -1.1606 -1.1557 -1.1508 -1.1459 -1.1409 -1.1359 -1.1309 -1.1259 -1.1209 -1.1158 -1.1108 -1.1057 -1.1006 -1.0955 -1.0904 -1.0853 -1.0802 -1.0751 -1.07 -1.065 -1.0599 -1.0549 -1.0498 -1.0448 -1.0398 -1.0348 -1.0299 -1.0249 -1.02 -1.0151 -1.0103 -1.0054 -1.0006 -0.9958 -0.99101 -0.98623 -0.98146 -0.97671 -0.97195 -0.96721 -0.96246 -0.95771 -0.95296 -0.9482 -0.94342 -0.93864 -0.93384 -0.92902 -0.92418 -0.91932 -0.91444 -0.90954 -0.90462 -0.89967 -0.8947 -0.88972 -0.88471 -0.87969 -0.87466 -0.86962 -0.86457 -0.85952 -0.85448 -0.84944 -0.8444 -0.83939 -0.83439 -0.82941 -0.82446 -0.81954 -0.81465 -0.8098 -0.80498 -0.8002 -0.79546 -0.79075 -0.78608 -0.78143 -0.77682 -0.77223 -0.76765 -0.76309 -0.75853 -0.75396 -0.74939 -0.74479 -0.74016 -0.7355 -0.73079 -0.72604 -0.72122 -0.71635 -0.71142 -0.70643 -0.70139 -0.6963 -0.69118 -0.68603 -0.68089 -0.67576 -0.6707 -0.66571 -0.66086 -0.65617 -0.65169 -0.64747 -0.64355 -0.64 -0.63685 -0.63414 -0.63191 -0.63017 -0.62894 -0.62818]
      | sbobj.Groups(1).Signals(3).Name = 'Position Angular z'
      | sbobj.Groups(1).Signals(3).XData = [0 0.15075 0.3015 0.45226 0.60301 0.75376 0.90451 1.0553 1.206 1.3568 1.5075 1.6583 1.809 1.9598 2.1105 2.2613 2.412 2.5628 2.7135 2.8643 3.015 3.1658 3.3165 3.4673 3.618 3.7688 3.9196 4.0703 4.2211 4.3718 4.5226 4.6733 4.8241 4.9748 5.1256 5.2763 5.4271 5.5778 5.7286 5.8793 6.0301 6.1808 6.3316 6.4823 6.6331 6.7838 6.9346 7.0853 7.2361 7.3869 7.5376 7.6884 7.8391 7.9899 8.1406 8.2914 8.4421 8.5929 8.7436 8.8944 9.0451 9.1959 9.3466 9.4974 9.6481 9.7989 9.9496 10.1 10.251 10.402 10.553 10.703 10.854 11.005 11.156 11.306 11.457 11.608 11.759 11.909 12.06 12.211 12.362 12.512 12.663 12.814 12.965 13.115 13.266 13.417 13.568 13.718 13.869 14.02 14.171 14.321 14.472 14.623 14.774 14.924 15.075 15.226 15.377 15.527 15.678 15.829 15.98 16.13 16.281 16.432 16.583 16.733 16.884 17.035 17.186 17.336 17.487 17.638 17.789 17.939 18.09 18.241 18.392 18.543 18.693 18.844 18.995 19.146 19.296 19.447 19.598 19.749 19.899 20.05 20.201 20.352 20.502 20.653 20.804 20.955 21.105 21.256 21.407 21.558 21.708 21.859 22.01 22.161 22.311 22.462 22.613 22.764 22.914 23.065 23.216 23.367 23.517 23.668 23.819 23.97 24.12 24.271 24.422 24.573 24.723 24.874 25.025 25.176 25.326 25.477 25.628 25.779 25.929 26.08 26.231 26.382 26.532 26.683 26.834 26.985 27.135 27.286 27.437 27.588 27.738 27.889 28.04 28.191 28.341 28.492 28.643 28.794 28.944 29.095 29.246 29.397 29.547 29.698 29.849 30]
      | sbobj.Groups(1).Signals(3).YData = [1.2662 2.3711 2.4881 2.554 2.6028 2.6413 2.6726 2.6985 2.7203 2.7387 2.7545 2.7681 2.7799 2.7901 2.799 2.8067 2.8135 2.8194 2.8246 2.8291 2.833 2.8364 2.8393 2.8419 2.8441 2.846 2.8476 2.849 2.8502 2.8513 2.8523 2.8532 2.854 2.8547 2.8554 2.8562 2.8569 2.8577 2.8584 2.8593 2.8601 2.861 2.8619 2.8629 2.8639 2.8649 2.866 2.8671 2.8681 2.8692 2.8703 2.8714 2.8725 2.8735 2.8745 2.8755 2.8764 2.8773 2.8781 2.8789 2.8796 2.8803 2.8809 2.8815 2.882 2.8825 2.8829 2.8832 2.8835 2.8838 2.8841 2.8843 2.8844 2.8846 2.8847 2.8849 2.885 2.8851 2.8852 2.8854 2.8855 2.8857 2.8859 2.8861 2.8863 2.8866 2.8869 2.8872 2.8876 2.888 2.8884 2.8889 2.8894 2.8899 2.8905 2.891 2.8916 2.8922 2.8928 2.8934 2.8941 2.8947 2.8953 2.8959 2.8965 2.8971 2.8977 2.8982 2.8987 2.8992 2.8997 2.9001 2.9005 2.9008 2.9011 2.9014 2.9016 2.9018 2.902 2.9021 2.9022 2.9023 2.9024 2.9024 2.9024 2.9024 2.9024 2.9024 2.9024 2.9024 2.9024 2.9024 2.9025 2.9025 2.9026 2.9027 2.9029 2.903 2.9032 2.9035 2.9038 2.9041 2.9044 2.9048 2.9052 2.9056 2.906 2.9065 2.907 2.9075 2.908 2.9085 2.9089 2.9094 2.9099 2.9103 2.9107 2.9111 2.9114 2.9117 2.912 2.9122 2.9123 2.9125 2.9125 2.9126 2.9125 2.9125 2.9124 2.9123 2.9121 2.912 2.9118 2.9117 2.9115 2.9114 2.9112 2.9111 2.9111 2.9111 2.9111 2.9112 2.9113 2.9114 2.9116 2.9118 2.912 2.9122 2.9124 2.9126 2.9128 2.9128 2.9129 2.9128 2.9128 2.9127 2.9126 2.9125 2.9127 2.9131]
      | sbobj.Groups(1).TimeRange = [0 30]
      | sbobj.Groups(2).Name = 'Position1'
      | sbobj.Groups(2).Signals(1).Name = 'Position Angular x'
      | sbobj.Groups(2).Signals(1).XData = [0 0.15075 0.3015 0.45226 0.60301 0.75376 0.90451 1.0553 1.206 1.3568 1.5075 1.6583 1.809 1.9598 2.1105 2.2613 2.412 2.5628 2.7135 2.8643 3.015 3.1658 3.3165 3.4673 3.618 3.7688 3.9196 4.0703 4.2211 4.3718 4.5226 4.6733 4.8241 4.9748 5.1256 5.2763 5.4271 5.5778 5.7286 5.8793 6.0301 6.1808 6.3316 6.4823 6.6331 6.7838 6.9346 7.0853 7.2361 7.3869 7.5376 7.6884 7.8391 7.9899 8.1406 8.2914 8.4421 8.5929 8.7436 8.8944 9.0451 9.1959 9.3466 9.4974 9.6481 9.7989 9.9496 10.1 10.251 10.402 10.553 10.703 10.854 11.005 11.156 11.306 11.457 11.608 11.759 11.909 12.06 12.211 12.362 12.512 12.663 12.814 12.965 13.115 13.266 13.417 13.568 13.718 13.869 14.02 14.171 14.321 14.472 14.623 14.774 14.924 15.075 15.226 15.377 15.527 15.678 15.829 15.98 16.13 16.281 16.432 16.583 16.733 16.884 17.035 17.186 17.336 17.487 17.638 17.789 17.939 18.09 18.241 18.392 18.543 18.693 18.844 18.995 19.146 19.296 19.447 19.598 19.749 19.899 20.05 20.201 20.352 20.502 20.653 20.804 20.955 21.105 21.256 21.407 21.558 21.708 21.859 22.01 22.161 22.311 22.462 22.613 22.764 22.914 23.065 23.216 23.367 23.517 23.668 23.819 23.97 24.12 24.271 24.422 24.573 24.723 24.874 25.025 25.176 25.326 25.477 25.628 25.779 25.929 26.08 26.231 26.382 26.532 26.683 26.834 26.985 27.135 27.286 27.437 27.588 27.738 27.889 28.04 28.191 28.341 28.492 28.643 28.794 28.944 29.095 29.246 29.397 29.547 29.698 29.849 30]
      | sbobj.Groups(2).Signals(1).YData = [-1.2662 -2.371 -2.4879 -2.5537 -2.6023 -2.6406 -2.6717 -2.6974 -2.7189 -2.7372 -2.7527 -2.7661 -2.7777 -2.7877 -2.7963 -2.8039 -2.8104 -2.8161 -2.821 -2.8252 -2.8289 -2.832 -2.8346 -2.8369 -2.8388 -2.8404 -2.8417 -2.8429 -2.8438 -2.8446 -2.8453 -2.8459 -2.8464 -2.8469 -2.8474 -2.8479 -2.8484 -2.8489 -2.8495 -2.85 -2.8507 -2.8513 -2.852 -2.8528 -2.8536 -2.8544 -2.8552 -2.856 -2.8569 -2.8577 -2.8586 -2.8594 -2.8602 -2.861 -2.8617 -2.8624 -2.863 -2.8636 -2.8641 -2.8646 -2.865 -2.8654 -2.8656 -2.8659 -2.866 -2.8662 -2.8662 -2.8662 -2.8662 -2.8661 -2.866 -2.8659 -2.8657 -2.8655 -2.8653 -2.8651 -2.8649 -2.8647 -2.8645 -2.8643 -2.8641 -2.8639 -2.8638 -2.8637 -2.8636 -2.8635 -2.8635 -2.8635 -2.8635 -2.8636 -2.8637 -2.8638 -2.864 -2.8641 -2.8643 -2.8646 -2.8648 -2.865 -2.8653 -2.8655 -2.8658 -2.866 -2.8662 -2.8664 -2.8666 -2.8668 -2.8669 -2.867 -2.8671 -2.8672 -2.8672 -2.8672 -2.8671 -2.867 -2.8668 -2.8666 -2.8664 -2.8662 -2.8659 -2.8655 -2.8652 -2.8648 -2.8644 -2.864 -2.8635 -2.863 -2.8626 -2.8621 -2.8616 -2.8612 -2.8607 -2.8602 -2.8598 -2.8594 -2.859 -2.8586 -2.8582 -2.8579 -2.8576 -2.8573 -2.8571 -2.8568 -2.8566 -2.8565 -2.8563 -2.8562 -2.8561 -2.856 -2.8559 -2.8558 -2.8557 -2.8556 -2.8555 -2.8554 -2.8553 -2.8551 -2.8549 -2.8547 -2.8544 -2.8541 -2.8538 -2.8534 -2.853 -2.8525 -2.852 -2.8514 -2.8508 -2.8502 -2.8495 -2.8487 -2.8479 -2.8471 -2.8463 -2.8454 -2.8445 -2.8436 -2.8428 -2.8419 -2.841 -2.8401 -2.8393 -2.8384 -2.8376 -2.8368 -2.8361 -2.8354 -2.8347 -2.834 -2.8334 -2.8328 -2.8322 -2.8317 -2.8312 -2.8307 -2.8303 -2.8299 -2.8295 -2.8292 -2.8291 -2.8291]
      | sbobj.Groups(2).Signals(2).Name = 'Position Angular y'
      | sbobj.Groups(2).Signals(2).XData = [0 0.15075 0.3015 0.45226 0.60301 0.75376 0.90451 1.0553 1.206 1.3568 1.5075 1.6583 1.809 1.9598 2.1105 2.2613 2.412 2.5628 2.7135 2.8643 3.015 3.1658 3.3165 3.4673 3.618 3.7688 3.9196 4.0703 4.2211 4.3718 4.5226 4.6733 4.8241 4.9748 5.1256 5.2763 5.4271 5.5778 5.7286 5.8793 6.0301 6.1808 6.3316 6.4823 6.6331 6.7838 6.9346 7.0853 7.2361 7.3869 7.5376 7.6884 7.8391 7.9899 8.1406 8.2914 8.4421 8.5929 8.7436 8.8944 9.0451 9.1959 9.3466 9.4974 9.6481 9.7989 9.9496 10.1 10.251 10.402 10.553 10.703 10.854 11.005 11.156 11.306 11.457 11.608 11.759 11.909 12.06 12.211 12.362 12.512 12.663 12.814 12.965 13.115 13.266 13.417 13.568 13.718 13.869 14.02 14.171 14.321 14.472 14.623 14.774 14.924 15.075 15.226 15.377 15.527 15.678 15.829 15.98 16.13 16.281 16.432 16.583 16.733 16.884 17.035 17.186 17.336 17.487 17.638 17.789 17.939 18.09 18.241 18.392 18.543 18.693 18.844 18.995 19.146 19.296 19.447 19.598 19.749 19.899 20.05 20.201 20.352 20.502 20.653 20.804 20.955 21.105 21.256 21.407 21.558 21.708 21.859 22.01 22.161 22.311 22.462 22.613 22.764 22.914 23.065 23.216 23.367 23.517 23.668 23.819 23.97 24.12 24.271 24.422 24.573 24.723 24.874 25.025 25.176 25.326 25.477 25.628 25.779 25.929 26.08 26.231 26.382 26.532 26.683 26.834 26.985 27.135 27.286 27.437 27.588 27.738 27.889 28.04 28.191 28.341 28.492 28.643 28.794 28.944 29.095 29.246 29.397 29.547 29.698 29.849 30]
      | sbobj.Groups(2).Signals(2).YData = [-1.5708 -1.5706 -1.5699 -1.5687 -1.5669 -1.5646 -1.5618 -1.5584 -1.5546 -1.5504 -1.5458 -1.5409 -1.5358 -1.5305 -1.525 -1.5195 -1.5138 -1.5082 -1.5025 -1.4969 -1.4914 -1.4859 -1.4804 -1.4751 -1.4698 -1.4647 -1.4596 -1.4546 -1.4496 -1.4447 -1.4399 -1.4351 -1.4303 -1.4255 -1.4208 -1.416 -1.4113 -1.4065 -1.4017 -1.3969 -1.392 -1.3871 -1.3822 -1.3772 -1.3722 -1.3672 -1.3621 -1.3569 -1.3518 -1.3466 -1.3414 -1.3361 -1.3309 -1.3256 -1.3204 -1.3151 -1.3098 -1.3046 -1.2993 -1.2941 -1.2889 -1.2837 -1.2785 -1.2734 -1.2683 -1.2632 -1.2582 -1.2532 -1.2482 -1.2432 -1.2383 -1.2334 -1.2285 -1.2236 -1.2187 -1.2139 -1.2091 -1.2042 -1.1994 -1.1946 -1.1898 -1.185 -1.1801 -1.1753 -1.1704 -1.1655 -1.1606 -1.1557 -1.1508 -1.1459 -1.1409 -1.1359 -1.1309 -1.1259 -1.1209 -1.1158 -1.1108 -1.1057 -1.1006 -1.0955 -1.0904 -1.0853 -1.0802 -1.0751 -1.07 -1.065 -1.0599 -1.0549 -1.0498 -1.0448 -1.0398 -1.0348 -1.0299 -1.0249 -1.02 -1.0151 -1.0103 -1.0054 -1.0006 -0.9958 -0.99101 -0.98623 -0.98146 -0.97671 -0.97195 -0.96721 -0.96246 -0.95771 -0.95296 -0.9482 -0.94342 -0.93864 -0.93384 -0.92902 -0.92418 -0.91932 -0.91444 -0.90954 -0.90462 -0.89967 -0.8947 -0.88972 -0.88471 -0.87969 -0.87466 -0.86962 -0.86457 -0.85952 -0.85448 -0.84944 -0.8444 -0.83939 -0.83439 -0.82941 -0.82446 -0.81954 -0.81465 -0.8098 -0.80498 -0.8002 -0.79546 -0.79075 -0.78608 -0.78143 -0.77682 -0.77223 -0.76765 -0.76309 -0.75853 -0.75396 -0.74939 -0.74479 -0.74016 -0.7355 -0.73079 -0.72604 -0.72122 -0.71635 -0.71142 -0.70643 -0.70139 -0.6963 -0.69118 -0.68603 -0.68089 -0.67576 -0.6707 -0.66571 -0.66086 -0.65617 -0.65169 -0.64747 -0.64355 -0.64 -0.63685 -0.63414 -0.63191 -0.63017 -0.62894 -0.62818]
      | sbobj.Groups(2).Signals(3).Name = 'Position Angular z'
      | sbobj.Groups(2).Signals(3).XData = [0 0.15075 0.3015 0.45226 0.60301 0.75376 0.90451 1.0553 1.206 1.3568 1.5075 1.6583 1.809 1.9598 2.1105 2.2613 2.412 2.5628 2.7135 2.8643 3.015 3.1658 3.3165 3.4673 3.618 3.7688 3.9196 4.0703 4.2211 4.3718 4.5226 4.6733 4.8241 4.9748 5.1256 5.2763 5.4271 5.5778 5.7286 5.8793 6.0301 6.1808 6.3316 6.4823 6.6331 6.7838 6.9346 7.0853 7.2361 7.3869 7.5376 7.6884 7.8391 7.9899 8.1406 8.2914 8.4421 8.5929 8.7436 8.8944 9.0451 9.1959 9.3466 9.4974 9.6481 9.7989 9.9496 10.1 10.251 10.402 10.553 10.703 10.854 11.005 11.156 11.306 11.457 11.608 11.759 11.909 12.06 12.211 12.362 12.512 12.663 12.814 12.965 13.115 13.266 13.417 13.568 13.718 13.869 14.02 14.171 14.321 14.472 14.623 14.774 14.924 15.075 15.226 15.377 15.527 15.678 15.829 15.98 16.13 16.281 16.432 16.583 16.733 16.884 17.035 17.186 17.336 17.487 17.638 17.789 17.939 18.09 18.241 18.392 18.543 18.693 18.844 18.995 19.146 19.296 19.447 19.598 19.749 19.899 20.05 20.201 20.352 20.502 20.653 20.804 20.955 21.105 21.256 21.407 21.558 21.708 21.859 22.01 22.161 22.311 22.462 22.613 22.764 22.914 23.065 23.216 23.367 23.517 23.668 23.819 23.97 24.12 24.271 24.422 24.573 24.723 24.874 25.025 25.176 25.326 25.477 25.628 25.779 25.929 26.08 26.231 26.382 26.532 26.683 26.834 26.985 27.135 27.286 27.437 27.588 27.738 27.889 28.04 28.191 28.341 28.492 28.643 28.794 28.944 29.095 29.246 29.397 29.547 29.698 29.849 30]
      | sbobj.Groups(2).Signals(3).YData = [1.2662 2.3711 2.4881 2.554 2.6028 2.6413 2.6726 2.6985 2.7203 2.7387 2.7545 2.7681 2.7799 2.7901 2.799 2.8067 2.8135 2.8194 2.8246 2.8291 2.833 2.8364 2.8393 2.8419 2.8441 2.846 2.8476 2.849 2.8502 2.8513 2.8523 2.8532 2.854 2.8547 2.8554 2.8562 2.8569 2.8577 2.8584 2.8593 2.8601 2.861 2.8619 2.8629 2.8639 2.8649 2.866 2.8671 2.8681 2.8692 2.8703 2.8714 2.8725 2.8735 2.8745 2.8755 2.8764 2.8773 2.8781 2.8789 2.8796 2.8803 2.8809 2.8815 2.882 2.8825 2.8829 2.8832 2.8835 2.8838 2.8841 2.8843 2.8844 2.8846 2.8847 2.8849 2.885 2.8851 2.8852 2.8854 2.8855 2.8857 2.8859 2.8861 2.8863 2.8866 2.8869 2.8872 2.8876 2.888 2.8884 2.8889 2.8894 2.8899 2.8905 2.891 2.8916 2.8922 2.8928 2.8934 2.8941 2.8947 2.8953 2.8959 2.8965 2.8971 2.8977 2.8982 2.8987 2.8992 2.8997 2.9001 2.9005 2.9008 2.9011 2.9014 2.9016 2.9018 2.902 2.9021 2.9022 2.9023 2.9024 2.9024 2.9024 2.9024 2.9024 2.9024 2.9024 2.9024 2.9024 2.9024 2.9025 2.9025 2.9026 2.9027 2.9029 2.903 2.9032 2.9035 2.9038 2.9041 2.9044 2.9048 2.9052 2.9056 2.906 2.9065 2.907 2.9075 2.908 2.9085 2.9089 2.9094 2.9099 2.9103 2.9107 2.9111 2.9114 2.9117 2.912 2.9122 2.9123 2.9125 2.9125 2.9126 2.9125 2.9125 2.9124 2.9123 2.9121 2.912 2.9118 2.9117 2.9115 2.9114 2.9112 2.9111 2.9111 2.9111 2.9111 2.9112 2.9113 2.9114 2.9116 2.9118 2.912 2.9122 2.9124 2.9126 2.9128 2.9128 2.9129 2.9128 2.9128 2.9127 2.9126 2.9125 2.9127 2.9131]
      | sbobj.Groups(2).TimeRange = [0 30]
  Subsystem : Subsystem
  Bus : Outport
  wires:
  Bus Creator/1 -> Bus/1
  Subsystem/3(Position Angular z) -> Bus Creator/3  "Position Angular z"
  Subsystem/2(Position Angular y) -> Bus Creator/2  "Position Angular y"
  Subsystem/1(Position Angular x) -> Bus Creator/1  "Position Angular x"
  FromWs/1 -> Subsystem/1(In1)

== system FreeFloatingNull/Signal Builder1 ==
  Bus Creator : BusCreator  Tag=Bus Creator  Inputs=6
  FromWs : FromWorkspace  Tag=STV FromWs  VariableName=tuvar  SampleTime=0
      SigBuilderData=|
      | common.afterFinalStr = 'Extrapolate'
      | common.sampleTime = 0
      | dataSet.timeRange = [0 30]
      | dataSet.name = 'Desired Velocities'
      | sbobj.Groups.Name = 'Desired Velocities'
      | sbobj.Groups.Signals(1).Name = 'Velocity Angular x'
      | sbobj.Groups.Signals(1).XData = [0 0.15075 0.3015 0.45226 0.60301 0.75376 0.90451 1.0553 1.206 1.3568 1.5075 1.6583 1.809 1.9598 2.1105 2.2613 2.412 2.5628 2.7135 2.8643 3.015 3.1658 3.3165 3.4673 3.618 3.7688 3.9196 4.0703 4.2211 4.3718 4.5226 4.6733 4.8241 4.9748 5.1256 5.2763 5.4271 5.5778 5.7286 5.8793 6.0301 6.1808 6.3316 6.4823 6.6331 6.7838 6.9346 7.0853 7.2361 7.3869 7.5376 7.6884 7.8391 7.9899 8.1406 8.2914 8.4421 8.5929 8.7436 8.8944 9.0451 9.1959 9.3466 9.4974 9.6481 9.7989 9.9496 10.1 10.251 10.402 10.553 10.703 10.854 11.005 11.156 11.306 11.457 11.608 11.759 11.909 12.06 12.211 12.362 12.512 12.663 12.814 12.965 13.115 13.266 13.417 13.568 13.718 13.869 14.02 14.171 14.321 14.472 14.623 14.774 14.924 15.075 15.226 15.377 15.527 15.678 15.829 15.98 16.13 16.281 16.432 16.583 16.733 16.884 17.035 17.186 17.336 17.487 17.638 17.789 17.939 18.09 18.241 18.392 18.543 18.693 18.844 18.995 19.146 19.296 19.447 19.598 19.749 19.899 20.05 20.201 20.352 20.502 20.653 20.804 20.955 21.105 21.256 21.407 21.558 21.708 21.859 22.01 22.161 22.311 22.462 22.613 22.764 22.914 23.065 23.216 23.367 23.517 23.668 23.819 23.97 24.12 24.271 24.422 24.573 24.723 24.874 25.025 25.176 25.326 25.477 25.628 25.779 25.929 26.08 26.231 26.382 26.532 26.683 26.834 26.985 27.135 27.286 27.437 27.588 27.738 27.889 28.04 28.191 28.341 28.492 28.643 28.794 28.944 29.095 29.246 29.397 29.547 29.698 29.849 30]
      | sbobj.Groups.Signals(1).YData = [0 -0.0018068 -0.0034031 -0.0047915 -0.0059792 -0.0069775 -0.0078002 -0.0084629 -0.0089823 -0.0093754 -0.0096591 -0.0098495 ... (200 elements, 1x200)]
      | sbobj.Groups.Signals(2).Name = 'Velocity Angular y'
      | sbobj.Groups.Signals(2).XData = [0 0.15075 0.3015 0.45226 0.60301 0.75376 0.90451 1.0553 1.206 1.3568 1.5075 1.6583 1.809 1.9598 2.1105 2.2613 2.412 2.5628 2.7135 2.8643 3.015 3.1658 3.3165 3.4673 3.618 3.7688 3.9196 4.0703 4.2211 4.3718 4.5226 4.6733 4.8241 4.9748 5.1256 5.2763 5.4271 5.5778 5.7286 5.8793 6.0301 6.1808 6.3316 6.4823 6.6331 6.7838 6.9346 7.0853 7.2361 7.3869 7.5376 7.6884 7.8391 7.9899 8.1406 8.2914 8.4421 8.5929 8.7436 8.8944 9.0451 9.1959 9.3466 9.4974 9.6481 9.7989 9.9496 10.1 10.251 10.402 10.553 10.703 10.854 11.005 11.156 11.306 11.457 11.608 11.759 11.909 12.06 12.211 12.362 12.512 12.663 12.814 12.965 13.115 13.266 13.417 13.568 13.718 13.869 14.02 14.171 14.321 14.472 14.623 14.774 14.924 15.075 15.226 15.377 15.527 15.678 15.829 15.98 16.13 16.281 16.432 16.583 16.733 16.884 17.035 17.186 17.336 17.487 17.638 17.789 17.939 18.09 18.241 18.392 18.543 18.693 18.844 18.995 19.146 19.296 19.447 19.598 19.749 19.899 20.05 20.201 20.352 20.502 20.653 20.804 20.955 21.105 21.256 21.407 21.558 21.708 21.859 22.01 22.161 22.311 22.462 22.613 22.764 22.914 23.065 23.216 23.367 23.517 23.668 23.819 23.97 24.12 24.271 24.422 24.573 24.723 24.874 25.025 25.176 25.326 25.477 25.628 25.779 25.929 26.08 26.231 26.382 26.532 26.683 26.834 26.985 27.135 27.286 27.437 27.588 27.738 27.889 28.04 28.191 28.341 28.492 28.643 28.794 28.944 29.095 29.246 29.397 29.547 29.698 29.849 30]
      | sbobj.Groups.Signals(2).YData = [0 -0.0022666 -0.0052246 -0.00859 -0.012137 -0.01569 -0.019115 -0.022315 -0.025222 -0.027794 -0.030007 -0.031856 -0.033348 -0.0345 -0.035335 -0.035883 -0.036178 -0.036253 -0.036144 -0.035884 -0.035509 -0.035047 -0.03453 -0.033981 -0.033425 -0.032881 -0.032366 -0.031893 -0.031474 -0.031115 -0.030823 -0.0306 -0.030446 -0.03036 -0.030339 -0.03038 -0.030476 -0.030621 -0.030809 -0.031031 -0.03128 -0.031549 -0.031829 -0.032114 -0.032396 -0.03267 -0.032929 -0.033168 -0.033383 -0.033571 -0.033727 -0.033851 -0.03394 -0.033995 -0.034015 -0.034001 -0.033954 -0.033876 -0.03377 -0.033638 -0.033484 -0.033311 -0.033123 -0.032923 -0.032715 -0.032504 -0.032292 -0.032084 -0.031883 -0.031691 -0.031513 -0.031351 -0.031207 -0.031082 -0.030979 -0.030899 -0.030841 -0.030808 -0.030797 -0.03081 -0.030845 -0.0309 -0.030975 -0.031068 -0.031176 -0.031297 -0.031429 -0.031568 -0.031714 -0.031861 -0.032009 -0.032154 -0.032293 -0.032425 -0.032546 -0.032654 -0.032747 -0.032824 -0.032884 -0.032924 -0.032945 -0.032945 -0.032924 -0.032883 -0.032822 -0.032742 -0.032644 -0.032528 -0.032398 -0.032254 -0.0321 -0.031936 -0.031767 -0.031593 -0.031419 -0.031246 -0.031078 -0.030917 -0.030765 -0.030626 -0.030501 -0.030393 -0.030302 -0.030232 -0.030182 -0.030155 -0.03015 -0.030167 -0.030207 -0.030268 -0.030351 -0.030452 -0.030571 -0.030705 -0.030852 -0.031009 -0.031172 -0.03134 -0.031507 -0.031672 -0.031829 -0.031975 -0.032108 -0.032222 -0.032316 -0.032386 -0.03243 -0.032445 -0.03243 -0.032383 -0.032304 -0.032194 -0.032052 -0.03188 -0.03168 -0.031456 -0.03121 -0.030948 -0.030673 -0.030391 -0.030109 -0.029833 -0.029569 -0.029325 -0.029107 -0.028922 -0.028776 -0.028675 -0.028625 -0.028629 -0.028689 -0.028808 -0.028985 -0.029218 -0.029501 -0.029828 -0.030189 -0.030572 -0.030961 -0.03134 -0.031686 -0.031977 -0.032187 -0.032287 -0.032248 -0.032039 -0.03163 -0.03099 -0.03009 -0.028908 -0.027423 -0.025625 -0.023511 -0.021094 -0.018401 -0.015482 -0.012411 -0.0092907 -0.0062639 -0.0035154]
      | sbobj.Groups.Signals(3).Name = 'Velocity Angular z'
      | sbobj.Groups.Signals(3).XData = [0 0.15075 0.3015 0.45226 0.60301 0.75376 0.90451 1.0553 1.206 1.3568 1.5075 1.6583 1.809 1.9598 2.1105 2.2613 2.412 2.5628 2.7135 2.8643 3.015 3.1658 3.3165 3.4673 3.618 3.7688 3.9196 4.0703 4.2211 4.3718 4.5226 4.6733 4.8241 4.9748 5.1256 5.2763 5.4271 5.5778 5.7286 5.8793 6.0301 6.1808 6.3316 6.4823 6.6331 6.7838 6.9346 7.0853 7.2361 7.3869 7.5376 7.6884 7.8391 7.9899 8.1406 8.2914 8.4421 8.5929 8.7436 8.8944 9.0451 9.1959 9.3466 9.4974 9.6481 9.7989 9.9496 10.1 10.251 10.402 10.553 10.703 10.854 11.005 11.156 11.306 11.457 11.608 11.759 11.909 12.06 12.211 12.362 12.512 12.663 12.814 12.965 13.115 13.266 13.417 13.568 13.718 13.869 14.02 14.171 14.321 14.472 14.623 14.774 14.924 15.075 15.226 15.377 15.527 15.678 15.829 15.98 16.13 16.281 16.432 16.583 16.733 16.884 17.035 17.186 17.336 17.487 17.638 17.789 17.939 18.09 18.241 18.392 18.543 18.693 18.844 18.995 19.146 19.296 19.447 19.598 19.749 19.899 20.05 20.201 20.352 20.502 20.653 20.804 20.955 21.105 21.256 21.407 21.558 21.708 21.859 22.01 22.161 22.311 22.462 22.613 22.764 22.914 23.065 23.216 23.367 23.517 23.668 23.819 23.97 24.12 24.271 24.422 24.573 24.723 24.874 25.025 25.176 25.326 25.477 25.628 25.779 25.929 26.08 26.231 26.382 26.532 26.683 26.834 26.985 27.135 27.286 27.437 27.588 27.738 27.889 28.04 28.191 28.341 28.492 28.643 28.794 28.944 29.095 29.246 29.397 29.547 29.698 29.849 30]
      | sbobj.Groups.Signals(3).YData = [0 0.00054192 0.00090485 0.0011364 0.0012753 0.0013522 0.0013906 0.0014082 0.0014177 0.0014277 0.0014432 0.0014672 0.0015001 0.0015414 0.0015895 0.001642 0.0016966 0.0017508 0.0018022 0.0018487 0.0018887 0.0019208 0.0019441 0.0019583 0.0019633 0.0019593 0.001947 0.0019273 0.0019012 0.0018699 0.0018349 0.0017974 0.0017589 0.0017206 0.0016839 0.00165 0.0016199 0.0015945 0.0015747 0.0015609 0.0015536 0.0015531 0.0015594 0.0015725 0.0015921 0.0016179 0.0016494 0.0016859 0.0017267 0.0017711 0.0018181 0.001867 0.0019168 0.0019667 0.0020158 0.0020633 0.0021083 0.0021503 0.0021887 0.0022228 0.0022524 0.002277 0.0022966 0.0023111 0.0023205 0.0023249 0.0023247 0.00232 0.0023115 0.0022996 0.0022848 0.0022678 0.0022493 0.0022298 0.0022102 0.0021911 0.0021732 0.0021571 0.0021435 0.0021328 0.0021257 0.0021224 0.0021234 0.002129 0.0021392 0.0021543 0.0021741 0.0021987 0.0022277 0.002261 0.0022981 0.0023387 0.0023823 0.0024282 0.0024759 0.0025248 0.0025741 0.0026231 0.0026711 0.0027175 0.0027615 0.0028026 0.0028401 0.0028734 0.0029022 0.002926 0.0029445 0.0029574 0.0029648 0.0029665 0.0029626 0.0029534 0.0029392 0.0029204 0.0028976 0.0028712 0.0028421 0.0028109 0.0027786 0.0027459 0.0027139 0.0026834 0.0026554 0.0026307 0.0026103 0.0025949 0.0025854 0.0025824 0.0025864 0.0025979 0.0026171 0.0026444 0.0026796 0.0027226 0.0027731 0.0028305 0.0028943 0.0029636 0.0030374 0.0031146 0.0031939 0.003274 0.0033534 0.0034307 0.0035042 0.0035724 0.0036338 0.003687 0.0037306 0.0037634 0.0037843 0.0037926 0.0037877 0.0037693 0.0037375 0.0036926 0.0036354 0.0035669 0.0034886 0.0034024 0.0033103 0.003215 0.0031191 0.0030257 0.002938 0.0028593 0.0027928 0.0027418 0.0027093 0.002698 0.0027102 0.0027474 0.0028108 0.0029002 0.0030149 0.0031528 0.0033106 0.0034836 0.0036659 0.0038501 0.0040275 0.004188 0.0043207 0.0044139 0.0044556 0.0044343 0.0043395 0.004163 0.0038999 0.0035504 0.0031216 0.0026293 0.0021014 0.0015799 0.0011252 0.00081917 0.00077016 0.0011172 0.0020355 0.0037422]
      | sbobj.Groups.Signals(4).Name = 'Velocity Linear x'
      | sbobj.Groups.Signals(4).XData = [0 0.15075 0.3015 0.45226 0.60301 0.75376 0.90451 1.0553 1.206 1.3568 1.5075 1.6583 1.809 1.9598 2.1105 2.2613 2.412 2.5628 2.7135 2.8643 3.015 3.1658 3.3165 3.4673 3.618 3.7688 3.9196 4.0703 4.2211 4.3718 4.5226 4.6733 4.8241 4.9748 5.1256 5.2763 5.4271 5.5778 5.7286 5.8793 6.0301 6.1808 6.3316 6.4823 6.6331 6.7838 6.9346 7.0853 7.2361 7.3869 7.5376 7.6884 7.8391 7.9899 8.1406 8.2914 8.4421 8.5929 8.7436 8.8944 9.0451 9.1959 9.3466 9.4974 9.6481 9.7989 9.9496 10.1 10.251 10.402 10.553 10.703 10.854 11.005 11.156 11.306 11.457 11.608 11.759 11.909 12.06 12.211 12.362 12.512 12.663 12.814 12.965 13.115 13.266 13.417 13.568 13.718 13.869 14.02 14.171 14.321 14.472 14.623 14.774 14.924 15.075 15.226 15.377 15.527 15.678 15.829 15.98 16.13 16.281 16.432 16.583 16.733 16.884 17.035 17.186 17.336 17.487 17.638 17.789 17.939 18.09 18.241 18.392 18.543 18.693 18.844 18.995 19.146 19.296 19.447 19.598 19.749 19.899 20.05 20.201 20.352 20.502 20.653 20.804 20.955 21.105 21.256 21.407 21.558 21.708 21.859 22.01 22.161 22.311 22.462 22.613 22.764 22.914 23.065 23.216 23.367 23.517 23.668 23.819 23.97 24.12 24.271 24.422 24.573 24.723 24.874 25.025 25.176 25.326 25.477 25.628 25.779 25.929 26.08 26.231 26.382 26.532 26.683 26.834 26.985 27.135 27.286 27.437 27.588 27.738 27.889 28.04 28.191 28.341 28.492 28.643 28.794 28.944 29.095 29.246 29.397 29.547 29.698 29.849 30]
      | sbobj.Groups.Signals(4).YData = [0 -0.0006469 -0.0019071 -0.0035651 -0.0054557 -0.0074534 -0.0094641 -0.011418 -0.013264 -0.014968 -0.016506 -0.017863 -0.019035 -0.020023 -0.020833 -0.021476 -0.021966 -0.02232 -0.022557 -0.022697 -0.022759 -0.022763 -0.022728 -0.022671 -0.022609 -0.022555 -0.022522 -0.022521 -0.022558 -0.02264 -0.022772 -0.022955 -0.023189 -0.023475 -0.023809 -0.024188 -0.024608 -0.025064 -0.02555 -0.026061 -0.026589 -0.02713 -0.027676 -0.028222 -0.028762 -0.029291 -0.029804 -0.030297 -0.030766 -0.031209 -0.031623 -0.032005 -0.032356 -0.032674 -0.03296 -0.033215 -0.03344 -0.033636 -0.033807 -0.033954 -0.034082 -0.034192 -0.034289 -0.034376 -0.034457 -0.034536 -0.034615 -0.034699 -0.034791 -0.034894 -0.03501 -0.035143 -0.035293 -0.035464 -0.035655 -0.035868 -0.036104 -0.036362 -0.036642 -0.036943 -0.037265 -0.037606 -0.037963 -0.038336 -0.038721 -0.039117 -0.03952 -0.039927 -0.040337 -0.040745 -0.04115 -0.041547 -0.041935 -0.042311 -0.042672 -0.043016 -0.043342 -0.043646 -0.043929 -0.044189 -0.044425 -0.044637 -0.044825 -0.044989 -0.04513 -0.045249 -0.045347 -0.045426 -0.045488 -0.045535 -0.045571 -0.045597 -0.045616 -0.045632 -0.045648 -0.045666 -0.04569 -0.045723 -0.045767 -0.045826 -0.045901 -0.045996 -0.046112 -0.04625 -0.046413 -0.0466 -0.046812 -0.04705 -0.047312 -0.047598 -0.047906 -0.048235 -0.048583 -0.048946 -0.049321 -0.049706 -0.050096 -0.050487 -0.050876 -0.051258 -0.051628 -0.051983 -0.052317 -0.052628 -0.05291 -0.053161 -0.053377 -0.053556 -0.053695 -0.053793 -0.053849 -0.053863 -0.053836 -0.053769 -0.053666 -0.053528 -0.053361 -0.05317 -0.052961 -0.05274 -0.052515 -0.052294 -0.052085 -0.051898 -0.05174 -0.051621 -0.051549 -0.051533 -0.051579 -0.051693 -0.051881 -0.052144 -0.052484 -0.0529 -0.053387 -0.053937 -0.054541 -0.055183 -0.055845 -0.056505 -0.057135 -0.057702 -0.058171 -0.0585 -0.058641 -0.058545 -0.058156 -0.057415 -0.05626 -0.054628 -0.052453 -0.049672 -0.046224 -0.042053 -0.037109 -0.031354 -0.024763 -0.017327 -0.0090607 9.2466e-16]
      | sbobj.Groups.Signals(5).Name = 'Velocity Linear y'
      | sbobj.Groups.Signals(5).XData = [0 0.15075 0.3015 0.45226 0.60301 0.75376 0.90451 1.0553 1.206 1.3568 1.5075 1.6583 1.809 1.9598 2.1105 2.2613 2.412 2.5628 2.7135 2.8643 3.015 3.1658 3.3165 3.4673 3.618 3.7688 3.9196 4.0703 4.2211 4.3718 4.5226 4.6733 4.8241 4.9748 5.1256 5.2763 5.4271 5.5778 5.7286 5.8793 6.0301 6.1808 6.3316 6.4823 6.6331 6.7838 6.9346 7.0853 7.2361 7.3869 7.5376 7.6884 7.8391 7.9899 8.1406 8.2914 8.4421 8.5929 8.7436 8.8944 9.0451 9.1959 9.3466 9.4974 9.6481 9.7989 9.9496 10.1 10.251 10.402 10.553 10.703 10.854 11.005 11.156 11.306 11.457 11.608 11.759 11.909 12.06 12.211 12.362 12.512 12.663 12.814 12.965 13.115 13.266 13.417 13.568 13.718 13.869 14.02 14.171 14.321 14.472 14.623 14.774 14.924 15.075 15.226 15.377 15.527 15.678 15.829 15.98 16.13 16.281 16.432 16.583 16.733 16.884 17.035 17.186 17.336 17.487 17.638 17.789 17.939 18.09 18.241 18.392 18.543 18.693 18.844 18.995 19.146 19.296 19.447 19.598 19.749 19.899 20.05 20.201 20.352 20.502 20.653 20.804 20.955 21.105 21.256 21.407 21.558 21.708 21.859 22.01 22.161 22.311 22.462 22.613 22.764 22.914 23.065 23.216 23.367 23.517 23.668 23.819 23.97 24.12 24.271 24.422 24.573 24.723 24.874 25.025 25.176 25.326 25.477 25.628 25.779 25.929 26.08 26.231 26.382 26.532 26.683 26.834 26.985 27.135 27.286 27.437 27.588 27.738 27.889 28.04 28.191 28.341 28.492 28.643 28.794 28.944 29.095 29.246 29.397 29.547 29.698 29.849 30]
      | sbobj.Groups.Signals(5).YData = [0 0.0019316 0.0034825 0.0047149 0.0056861 0.0064464 0.0070393 0.007501 0.0078612 0.0081436 0.0083667 0.0085448 0.0086886 0.008806 0.0089029 0.0089833 0.0090503 0.009106 0.0091518 0.009189 0.0092184 0.0092408 0.0092568 0.0092671 0.0092721 0.0092726 0.0092691 0.0092623 0.0092527 0.009241 0.009228 0.0092142 0.0092004 0.0091874 0.0091758 0.0091665 0.0091601 0.0091573 0.009159 0.0091657 0.0091781 0.0091968 0.0092222 0.0092549 0.009295 0.0093429 0.0093987 0.0094623 0.0095338 0.0096129 0.0096992 0.0097925 0.0098921 0.0099974 0.010108 0.010223 0.010341 0.010462 0.010585 0.010708 0.010832 0.010954 0.011075 0.011193 0.011307 0.011417 0.011522 0.011621 0.011714 0.011799 0.011878 0.011949 0.012012 0.012067 0.012114 0.012153 0.012184 0.012207 0.012223 0.012232 0.012235 0.012233 0.012225 0.012213 0.012197 0.012179 0.012159 0.012138 0.012117 0.012098 0.012081 0.012066 0.012056 0.012051 0.012051 0.012058 0.012073 0.012095 0.012125 0.012165 0.012214 0.012273 0.012341 0.012419 0.012506 0.012603 0.012709 0.012823 0.012946 0.013075 0.013211 0.013353 0.013499 0.013649 0.013802 0.013955 0.014109 0.014261 0.01441 0.014556 0.014697 0.014832 0.014959 0.015077 0.015186 0.015285 0.015372 0.015448 0.015511 0.015561 0.015598 0.015622 0.015633 0.015632 0.015619 0.015594 0.015559 0.015514 0.015461 0.015402 0.015337 0.015269 0.015199 0.015129 0.015062 0.014999 0.014943 0.014895 0.014858 0.014834 0.014825 0.014833 0.01486 0.014906 0.014974 0.015065 0.015179 0.015317 0.01548 0.015667 0.015877 0.01611 0.016365 0.01664 0.016933 0.017241 0.017561 0.017891 0.018227 0.018564 0.018899 0.019228 0.019544 0.019845 0.020125 0.020378 0.0206 0.020786 0.02093 0.021027 0.021072 0.021059 0.020983 0.020838 0.020618 0.020316 0.019926 0.019438 0.018845 0.018135 0.017296 0.016314 0.01517 0.013843 0.012306 0.010527 0.0084644 0.0060676 0.0032728 -5.8634e-16]
      | sbobj.Groups.Signals(6).Name = 'Velocity Linear z'
      | sbobj.Groups.Signals(6).XData = [0 0.15075 0.3015 0.45226 0.60301 0.75376 0.90451 1.0553 1.206 1.3568 1.5075 1.6583 1.809 1.9598 2.1105 2.2613 2.412 2.5628 2.7135 2.8643 3.015 3.1658 3.3165 3.4673 3.618 3.7688 3.9196 4.0703 4.2211 4.3718 4.5226 4.6733 4.8241 4.9748 5.1256 5.2763 5.4271 5.5778 5.7286 5.8793 6.0301 6.1808 6.3316 6.4823 6.6331 6.7838 6.9346 7.0853 7.2361 7.3869 7.5376 7.6884 7.8391 7.9899 8.1406 8.2914 8.4421 8.5929 8.7436 8.8944 9.0451 9.1959 9.3466 9.4974 9.6481 9.7989 9.9496 10.1 10.251 10.402 10.553 10.703 10.854 11.005 11.156 11.306 11.457 11.608 11.759 11.909 12.06 12.211 12.362 12.512 12.663 12.814 12.965 13.115 13.266 13.417 13.568 13.718 13.869 14.02 14.171 14.321 14.472 14.623 14.774 14.924 15.075 15.226 15.377 15.527 15.678 15.829 15.98 16.13 16.281 16.432 16.583 16.733 16.884 17.035 17.186 17.336 17.487 17.638 17.789 17.939 18.09 18.241 18.392 18.543 18.693 18.844 18.995 19.146 19.296 19.447 19.598 19.749 19.899 20.05 20.201 20.352 20.502 20.653 20.804 20.955 21.105 21.256 21.407 21.558 21.708 21.859 22.01 22.161 22.311 22.462 22.613 22.764 22.914 23.065 23.216 23.367 23.517 23.668 23.819 23.97 24.12 24.271 24.422 24.573 24.723 24.874 25.025 25.176 25.326 25.477 25.628 25.779 25.929 26.08 26.231 26.382 26.532 26.683 26.834 26.985 27.135 27.286 27.437 27.588 27.738 27.889 28.04 28.191 28.341 28.492 28.643 28.794 28.944 29.095 29.246 29.397 29.547 29.698 29.849 30]
      | sbobj.Groups.Signals(6).YData = [0 0.0063472 0.013725 0.021607 0.029579 0.037322 0.044602 0.051251 0.057163 0.06228 0.066581 0.070078 0.072807 0.074819 0.076181 0.076964 0.077246 0.077103 0.076612 0.075845 0.074871 0.073751 0.072542 0.071292 0.070045 0.068835 0.067693 0.06664 0.065694 0.064866 0.064164 0.06359 0.063142 0.062816 0.062605 0.062498 0.062484 0.062552 0.062686 0.062875 0.063102 0.063355 0.06362 0.063885 0.064138 0.064368 0.064567 0.064726 0.064839 0.064901 0.064907 0.064856 0.064745 0.064576 0.064349 0.064066 0.063731 0.063347 0.062919 0.062452 0.061951 0.061423 0.060873 0.060307 0.059732 0.059153 0.058576 0.058006 0.057449 0.056909 0.05639 0.055895 0.055429 0.054992 0.054587 0.054215 0.053876 0.053572 0.0533 0.05306 0.05285 0.052669 0.052514 0.052382 0.052269 0.052173 0.05209 0.052015 0.051947 0.051879 0.05181 0.051734 0.051649 0.051551 0.051438 0.051306 0.051153 0.050977 0.050776 0.05055 0.050296 0.050015 0.049706 0.04937 0.049008 0.048621 0.04821 0.047777 0.047325 0.046855 0.04637 0.045874 0.045369 0.044858 0.044344 0.043831 0.043322 0.04282 0.042328 0.041849 0.041385 0.040939 0.040513 0.040109 0.039728 0.039371 0.03904 0.038734 0.038453 0.038197 0.037965 0.037755 0.037566 0.037396 0.037241 0.0371 0.036969 0.036845 0.036723 0.036602 0.036476 0.036341 0.036195 0.036034 0.035853 0.03565 0.035422 0.035166 0.034881 0.034563 0.034212 0.033828 0.03341 0.032959 0.032476 0.031962 0.031422 0.030856 0.03027 0.029668 0.029053 0.028432 0.027811 0.027194 0.026589 0.026001 0.025437 0.024902 0.024402 0.023943 0.023527 0.023159 0.022841 0.022573 0.022354 0.022184 0.022056 0.021965 0.021903 0.021858 0.021819 0.02177 0.021694 0.021574 0.021389 0.021119 0.02074 0.020232 0.019573 0.018744 0.017726 0.016506 0.015074 0.013425 0.011564 0.0095037 0.007268 0.0048968 0.0024476 -3.505e-15]
      | sbobj.Groups.TimeRange = [0 30]
  Subsystem : Subsystem
  Bus : Outport
  wires:
  Bus Creator/1 -> Bus/1
  Subsystem/6(Velocity Linear z) -> Bus Creator/6  "Velocity Linear z"
  Subsystem/5(Velocity Linear y) -> Bus Creator/5  "Velocity Linear y"
  Subsystem/4(Velocity Linear x) -> Bus Creator/4  "Velocity Linear x"
  Subsystem/3(Velocity Angular z) -> Bus Creator/3  "Velocity Angular z"
  Subsystem/2(Velocity Angular y) -> Bus Creator/2  "Velocity Angular y"
  Subsystem/1(Velocity Angular x) -> Bus Creator/1  "Velocity Angular x"
  FromWs/1 -> Subsystem/1(In1)

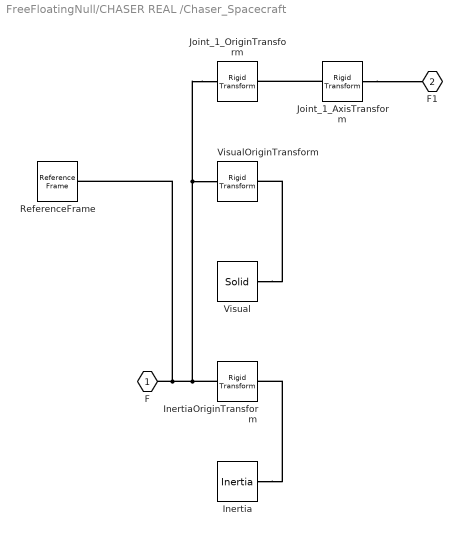
== system FreeFloatingNull/CHASER REAL /Chaser_Spacecraft ==
  Inertia : sm_lib/Body Elements/Inertia  InertiaType=Custom  Mass=1580  MassUnits=kg  CenterOfMass=[0, 0, 0]  CenterOfMassUnits=m  MomentsOfInertia=[1481.2, 1481.2, 592.4763]  MomentsOfInertiaUnits=kg*m^2  ProductsOfInertia=[0, 0, 0]  ProductsOfInertiaUnits=kg*m^2  GraphicType=None  MarkerShape=Inertia  MarkerSize=20  GraphicVisPropType=SimpleVisualProperties  GraphicDiffuseColor=[0.5 0.5 0.5]  GraphicSpecularColor=[0.5 0.5 0.5 1.0]  GraphicAmbientColor=[0.15 0.15 0.15 1.0]  GraphicEmissiveColor=[0.0 0.0 0.0 1.0]  GraphicShininess=75  GraphicOpacity=1.0
  InertiaOriginTransform : sm_lib/Frames and Transforms/Rigid Transform  TranslationMethod=Cartesian  TranslationStandardOffset=0  TranslationLengthUnit=m  TranslationStandardAxis=+Z  TranslationCartesianOffset=[0, 0, 0]  TranslationROffset=0  TranslationROffsetUnits=m  TranslationZOffset=0  TranslationZOffsetUnits=m  TranslationThetaOffset=0  TranslationThetaOffsetUnits=deg  RotationMethod=RotationSequence  RotationAngleUnits=deg  RotationStandardAxis=+Z  RotationAngle=0.0  RotationArbitraryAxis=[0 0 1]  FollAlignAxisA=+X  BaseAlignAxisA=+Y  FollAlignAxisB=+Y  BaseAlignAxisB=+Z  RotationSequenceAxes=BaseAxes  RotationSequence=XYZ  RotationSequenceAngles=[0, 0, 0]  RotationSequenceAnglesUnits=rad  RotationMatrix=[1 0 0; 0 1 0; 0 0 1]
  Joint_1_AxisTransform : sm_lib/Frames and Transforms/Rigid Transform  TranslationMethod=Cartesian  TranslationStandardOffset=0  TranslationLengthUnit=m  TranslationStandardAxis=+Z  TranslationCartesianOffset=[0, 0, 0]  TranslationROffset=0  TranslationROffsetUnits=m  TranslationZOffset=0  TranslationZOffsetUnits=m  TranslationThetaOffset=0  TranslationThetaOffsetUnits=deg  RotationMethod=ArbitraryAxis  RotationAngleUnits=rad  RotationStandardAxis=+Z  RotationAngle=0  RotationArbitraryAxis=[1, 0, 0]  FollAlignAxisA=+X  BaseAlignAxisA=+Y  FollAlignAxisB=+Y  BaseAlignAxisB=+Z  RotationSequenceAxes=FollowerAxes  RotationSequence=XYX  RotationSequenceAngles=[0 0 0]  RotationSequenceAnglesUnits=deg  RotationMatrix=[1 0 0; 0 1 0; 0 0 1]
  Joint_1_OriginTransform : sm_lib/Frames and Transforms/Rigid Transform  TranslationMethod=Cartesian  TranslationStandardOffset=0  TranslationLengthUnit=m  TranslationStandardAxis=+Z  TranslationCartesianOffset=[0.75, 0, 1.4]  TranslationROffset=0  TranslationROffsetUnits=m  TranslationZOffset=0  TranslationZOffsetUnits=m  TranslationThetaOffset=0  TranslationThetaOffsetUnits=deg  RotationMethod=RotationSequence  RotationAngleUnits=deg  RotationStandardAxis=+Z  RotationAngle=0.0  RotationArbitraryAxis=[0 0 1]  FollAlignAxisA=+X  BaseAlignAxisA=+Y  FollAlignAxisB=+Y  BaseAlignAxisB=+Z  RotationSequenceAxes=BaseAxes  RotationSequence=XYZ  RotationSequenceAngles=[3.1416, -1.570796, 0]  RotationSequenceAnglesUnits=rad  RotationMatrix=[1 0 0; 0 1 0; 0 0 1]
  ReferenceFrame : sm_lib/Frames and Transforms/Reference Frame
  Visual : sm_lib/Body Elements/Solid  InertiaType=Custom  Mass=0  MassUnits=kg  CenterOfMass=[0, 0, 0]  CenterOfMassUnits=m  MomentsOfInertia=[0, 0, 0]  MomentsOfInertiaUnits=kg*m^2  ProductsOfInertia=[0, 0, 0]  ProductsOfInertiaUnits=kg*m^2  BasedOnType=Density  Density=1000  DensityUnits=kg/m^3  DoExposeReferenceFrame=on  SerializedFrames=<Frames/>  GraphicType=FromGeometry  MarkerShape=Sphere  MarkerSize=10  GraphicVisPropType=SimpleVisualProperties  GraphicDiffuseColor=[0.2, 0.2, 0.2]  GraphicSpecularColor=[0.5 0.5 0.5 1.0]  GraphicAmbientColor=[0.15 0.15 0.15 1.0]  GraphicEmissiveColor=[0.0 0.0 0.0 1.0]  GraphicShininess=75  GraphicOpacity=1  GeometryShape=Brick  RectangleSize=[1 1]  RectangleSizeUnits=m  BrickDimensions=[1.5, 1.5, 3]  BrickDimensionUnits=m  CylinderRadius=1  CylinderRadiusUnits=m  CylinderLength=1  CylinderLengthUnits=m  SphereRadius=1  SphereRadiusUnits=m  EllipsoidRadii=[1 1 1]  EllipsoidRadiiUnits=m  ExtrusionCrossSection=[1 1; -1 1; -1 -1; 1 -1]  ExtrusionCrossSectionUnits=m  ExtrusionLength=1  ExtrusionLengthUnits=m  PolygonNumSides=3  PolygonOuterRadius=1  PolygonOuterRadiusUnits=m  ExtGeomFileType=STEP  ExtGeomFileUnits=m  RevolutionCrossSection=[1 1; 1 -1; 2 -1; 2 1]  RevolutionCrossSectionUnits=m  RevolutionExtent=Full  RevolutionAngle=180  RevolutionAngleUnits=deg
  VisualOriginTransform : sm_lib/Frames and Transforms/Rigid Transform  TranslationMethod=Cartesian  TranslationStandardOffset=0  TranslationLengthUnit=m  TranslationStandardAxis=+Z  TranslationCartesianOffset=[0, 0, 0]  TranslationROffset=0  TranslationROffsetUnits=m  TranslationZOffset=0  TranslationZOffsetUnits=m  TranslationThetaOffset=0  TranslationThetaOffsetUnits=deg  RotationMethod=RotationSequence  RotationAngleUnits=deg  RotationStandardAxis=+Z  RotationAngle=0.0  RotationArbitraryAxis=[0 0 1]  FollAlignAxisA=+X  BaseAlignAxisA=+Y  FollAlignAxisB=+Y  BaseAlignAxisB=+Z  RotationSequenceAxes=BaseAxes  RotationSequence=XYZ  RotationSequenceAngles=[0, 0, 0]  RotationSequenceAnglesUnits=rad  RotationMatrix=[1 0 0; 0 1 0; 0 0 1]
  F : PMIOPort  Side=Left
  F1 : PMIOPort  Port=2  Side=Right
  connections:
  Inertia/RConn1 -- InertiaOriginTransform/RConn1
  Joint_1_AxisTransform/RConn1 -- F1/RConn1
  Joint_1_AxisTransform/LConn1 -- Joint_1_OriginTransform/RConn1
  Joint_1_OriginTransform/LConn1 -- InertiaOriginTransform/LConn1 -- ReferenceFrame/RConn1 -- F/RConn1 -- VisualOriginTransform/LConn1
  Visual/RConn1 -- VisualOriginTransform/RConn1
